simulink model "ENV"  (R2024b)
settings: Solver=FixedStepDiscrete  StartTime=0.0  StopTime=1  FixedStep=0.001  RelTol=1e-3  EnableMultiTasking=on
PreLoadFcn:
  | load('CAN_MESSAGE_bus.mat');
libraries: stm32blockslib x62, canmsglib x28, simulink x6, stm32f4xxblockslib x3
(part 1 of 5)
settings Model: DataDictionary=Master_Dictionary.sldd  EnableAccessToBaseWorkspace=off  STM32="{\"DigitalPortRead\":{\"ID\":\"ENV:1737\"},\"SPIControllerTransfer\":[{\"ID\":\"ENV:2145\"},{\"ID\":\"ENV:2146\"},{\"ID\":\"ENV:2312\"},{\"ID\":\"ENV:2313\"},{\"ID\":\"ENV:2314\"},{\"ID\":\"ENV:1806\"},{\"ID\":\"ENV:1805\"},{\"ID\":\"ENV:2392\"},{\"ID\":\"ENV:2393\"},{\"ID\":\"ENV:2419\"},{\"ID\":\"ENV:2421\"},{\"ID\":\"ENV:2432\"},{\"ID\":\"ENV:2439\"},{\"ID\":\"ENV:2451\"},{\"ID\":\"ENV:2458\"},{\"ID\":\"ENV:1834\"},{\"ID\":\"ENV:1835\"},{\"ID\":\"ENV:1851\"},{\"ID\":\"ENV:1852\"},{\"ID\":\"ENV:1875\"},{\"ID\":\"ENV:1876\"},{\"ID\":\"ENV:1893\"},{\"ID\":\"ENV:1894\"},{\"ID\":\"ENV:1915\"},{\"ID\":\"ENV:1916\"},{\"ID\":\"ENV:1940\"},{\"ID\":\"ENV:1941\"},{\"ID\":\"ENV:1960\"},{\"ID\":\"ENV:1961\"},{\"ID\":\"ENV:1982\"},{\"ID\":\"ENV:1983\"},{\"ID\":\"ENV:2003\"},{\"ID\":\"ENV:2004\"},{\"ID\":\"ENV:2024\"},{\"ID\":\"ENV:2025\"},{\"ID\":\"ENV:2071\"},{\"ID\":\"ENV:2072\"},{\"ID\":\"ENV:2091\"},{\"ID\":\"ENV:2092\"},{\"ID\":\"ENV:2117\"},{\"ID\":\"ENV:2118\"},{\"ID\":\"ENV:2169\"},{\"ID\":\"ENV:2170\"},{\"ID\":\"ENV:2191\"},{\"ID\":\"ENV:2192\"},{\"ID\":\"ENV:2213\"},{\"ID\":\"ENV:2214\"},{\"ID\":\"ENV:2234\"},{\"ID\":\"ENV:2235\"},{\"ID\":\"ENV:2254\"},{\"ID\":\"ENV:2255\"},{\"ID\":\"ENV:2522\"},{\"ID\":\"ENV:2521\"},{\"ID\":\"ENV:2520\"},{\"ID\":\"ENV:2519\"},{\"ID\":\"ENV:2518\"},{\"ID\":\"ENV:2517\"},{\"ID\":\"ENV:2516\"},{\"ID\":\"ENV:2515\"},{\"ID\":\"ENV:2549\"},{\"ID\":\"ENV:2550\"},{\"ID\":\"ENV:2555\"}],\"DigitalPortWrite\":[{\"ID\":\"ENV:2350\"},{\"ID\":\"ENV:2481\"}]}"  Creator=oxbro  LastModifiedBy=oxbro
settings SolverCC: AlgebraicLoopSolver=TrustRegion
settings DataIOCC: ReturnWorkspaceOutputs=off
settings OptimizationCC: DefaultParameterBehavior=Inlined  EnhancedBackFolding=on  PassReuseOutputArgsAs=Individual arguments  ZeroExternalMemoryAtStartup=off  ZeroInternalMemoryAtStartup=off  MaxStackSize=512  OptimizeBlockOrder=speed  DifferentSizesBufferReuse=on  OptimizationCustomize=off  EfficientTunableParamExpr=on
settings DebuggingCC: ParameterTunabilityLossMsg=error  UnconnectedInputMsg=warning  UnconnectedOutputMsg=warning  UnconnectedLineMsg=warning  ArithmeticOperatorsInVariantConditions=warning
settings HardwareCC: ProdBitPerPointer=32  ProdBitPerSizeT=32  ProdBitPerPtrDiffT=32  ProdLargestAtomicInteger=Long  ProdLargestAtomicFloat=Double  ProdWordSize=32  ProdLongLongMode=on  ProdHWDeviceType=ARM Compatible->ARM Cortex-M
settings ModelReferenceCC: EnableRefExpFcnMdlSchedulingChecks=on
settings SFSimCC: MATLABDynamicMemAlloc=off  CustomCodeUndefinedFunction=UseInterfaceOnly
settings RTWCC: Description=Embedded Coder  SystemTargetFile=ert.tlc  HardwareBoard=STM32H7xx Based (Single-core)  TemplateMakefile=ert_default_tmf  CustomHeaderCode="#include \"stm32h7xx_ll_tim.h\""  CustomInitializer=LL_TIM_EnableCounter(TIM2);  Toolchain=GNU Tools for ARM Embedded Processors  GPUComputeCapability=3.5
settings CodeAppCC: ForceParamTrailComments=on  IgnoreCustomStorageClasses=off  OperatorAnnotations=on  SimulinkDataObjDesc=on  SFDataObjDesc=on  InsertBlockDesc=on
settings ERTTargetCC: TargetLangStandard=C99 (ISO)  CodeReplacementLibrary=ARM Cortex-M  ExtModeTransport=3  ExtModeStaticAlloc=on  ExtModeStaticAllocSize=2048  ExtModeMexFile=ext_xcp  ExtModeIntrfLevel=Level2 - Open

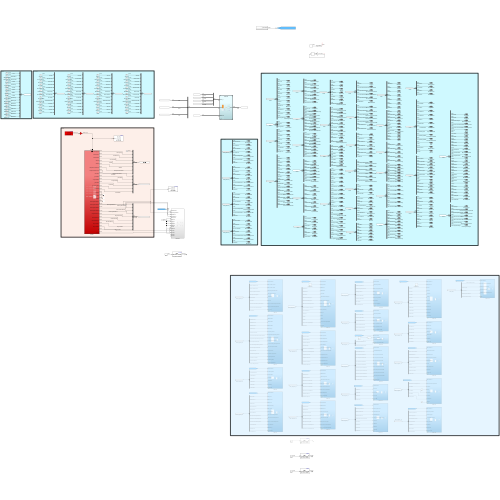
[thumbnail: Simulink's stored preview of the top-level diagram]
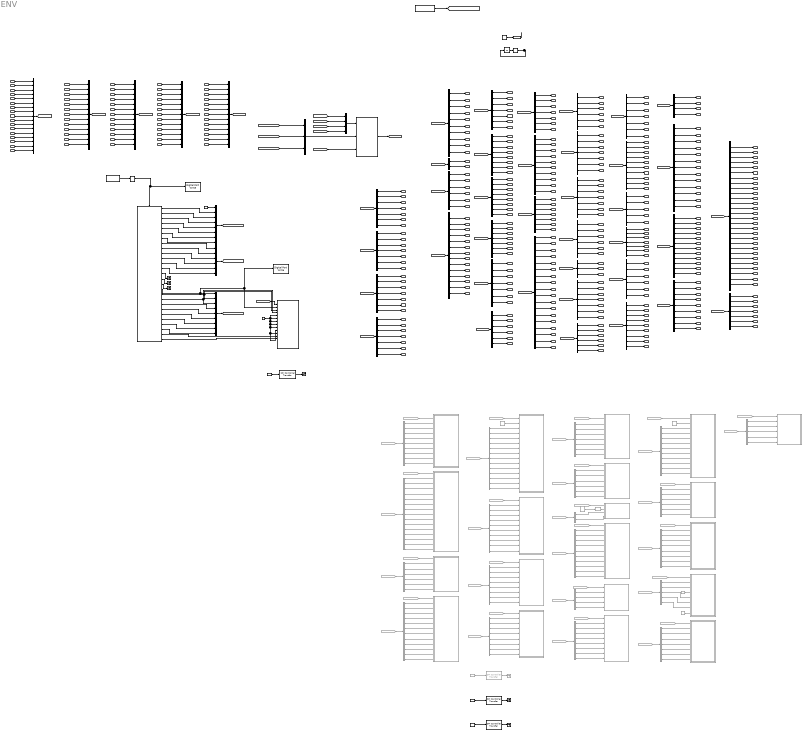
== system ENV ==
  note: CAN3
  note: CAN 1&2
  note: CAN4
  note: CAN1&2
  note: CAN3
  note: CAN3
  nMotorRL : Inport
  BInvDCOnRLIn : Inport  Port=2
  BInvErrorRL : Inport  Port=3
  BInvOnRLIn : Inport  Port=4
  BInvQuitDcOnRL : Inport  Port=5
  BQuitInvOnRL : Inport  Port=6
  BInvSysReadyRL : Inport  Port=7
  BInvWarnRL : Inport  Port=8
  MMotorMeasuredRL : Inport  Port=9
  NInvDTCRL : Inport  Port=10
  TMotorRL : Inport  Port=11
  VDCInvRL : Inport  Port=12
  TInvRL : Inport  Port=13
  nMotorRR : Inport  Port=14
  BInvDCOnRRIn : Inport  Port=15
  BInvErrorRR : Inport  Port=16
  BInvOnRRIn : Inport  Port=17
  BInvQuitDcOnRR : Inport  Port=18
  BQuitInvOnRR : Inport  Port=19
  BInvSysReadyRR : Inport  Port=20
  BInvWarnRR : Inport  Port=21
  MMotorMeasuredRR : Inport  Port=22
  NInvDTCRR : Inport  Port=23
  TMotorRR : Inport  Port=24
  VDCInvRR : Inport  Port=25
  TInvRR : Inport  Port=26
  nMotorFL : Inport  Port=27
  BInvDCOnFLIn : Inport  Port=28
  BInvErrorFL : Inport  Port=29
  BInvOnFLIn : Inport  Port=30
  BInvQuitDcOnFL : Inport  Port=31
  BQuitInvOnFL : Inport  Port=32
  BInvSysReadyFL : Inport  Port=33
  BInvWarnFL : Inport  Port=34
  MMotorMeasuredFL : Inport  Port=35
  NInvDTCFL : Inport  Port=36
  TMotorFL : Inport  Port=37
  VDCInvFL : Inport  Port=38
  TInvFL : Inport  Port=39
  nMotorFR : Inport  Port=40
  BInvDCOnFRIn : Inport  Port=41
  BInvErrorFR : Inport  Port=42
  BInvOnFRIn : Inport  Port=43
  BInvQuitDcOnFR : Inport  Port=44
  BQuitInvOnFR : Inport  Port=45
  BInvSysReadyFR : Inport  Port=46
  BInvWarnFR : Inport  Port=47
  MMotorMeasuredFR : Inport  Port=48
  NInvDTCFR : Inport  Port=49
  TMotorFR : Inport  Port=50
  VDCInvFR : Inport  Port=51
  TInvFR : Inport  Port=52
  IIVTS : Inport  Port=53
  IBMSHallEffect : Inport  Port=54
  VDCAccumulator : Inport  Port=55
  TCellMin : Inport  Port=56
  VCellAverage : Inport  Port=57
  VCellMax : Inport  Port=58
  TCellMax : Inport  Port=59
  IBMSDCL : Inport  Port=60
  VCellMin : Inport  Port=61
  RCellAverage : Inport  Port=62
  BBalancingOn : Inport  Port=63
  BBMSP0A0C : Inport  Port=64  OutDataTypeStr=boolean
  BBMSP0A0E : Inport  Port=65
  BBMSP0A10 : Inport  Port=66
  BBMSP0A80 : Inport  Port=67
  BBMSP0AC0 : Inport  Port=68
  BBMSP0AFA : Inport  Port=69
  Bus Creator : BusCreator  Inputs=3  OutDataTypeStr=Bus: CAN3Bus
  Bus Creator14 : BusCreator  Inputs=13  OutDataTypeStr=Bus: InverterFL
  Bus Creator15 : BusCreator  Inputs=13  OutDataTypeStr=Bus: InverterFR
  Bus Creator17 : BusCreator  Inputs=13  OutDataTypeStr=Bus: InverterRL
  Bus Creator18 : BusCreator  Inputs=17  OutDataTypeStr=Bus: BMS
  Bus Creator19 : BusCreator  Inputs=13  OutDataTypeStr=Bus: InverterRR
  Bus Creator2 : BusCreator  Inputs=8  OutDataTypeStr=Bus: DDU7
  Bus Creator3 : BusCreator  Inputs=6  OutDataTypeStr=Bus: IMU
      settings: InheritFromInputs=off
  Bus Creator4 : BusCreator  Inputs=9  OutDataTypeStr=Bus: STW
  Bus Selector : BusSelector  OutputSignals=TorqueControl.MFLFinal,TorqueControl.MFRFinal,TorqueControl.MRLFinal,TorqueControl.MRRFinal,BMSSignals.IIVTS,Systems.PActual,Systems.BBrakeError,Systems.BThrottleError,Systems.BOverpower,Limitations.BDischargeAllowed
  Bus Selector1 : BusSelector  OutputSignals=Systems.vChassis,Systems.PEnergyMeter
  Bus Selector10 : BusSelector  OutputSignals=TorqueControl.MTotalRequested,TorqueControl.rSlipRatioOptimal,TorqueControl.aCamberFL,TorqueControl.aCamberFR,TorqueControl.aCamberRL,TorqueControl.aCamberRR,TorqueControl.FTotalLateralLoadTransfer
  Bus Selector11 : BusSelector  OutputSignals=Systems.BTVOnEM,Systems.BTVOnOW,Systems.BDrivetrainCoolingOn,Systems.BDrivetrainCoolingOnEM,Systems.BDrivetrainCoolingOnOW,Systems.BTCOn,Systems.BTCOnEM,Systems.BTCOnOW,Systems.BEMSOn,Systems.BEMSOnEM,Systems.BEMSOnOW,Systems.BSpinningModeOn,Systems.BSpinningModeOnEM,Systems.BSpinningModeOnOW,Systems.rSOE,BMSSignals.BBalancingOn,BMSSignals.BBMSP0A0C,BMSSignals.BBMSP0A0E,BMSSignals.BBMSP0A10,BMSSignals.BBMSP0A80,BMSSignals.BBMSP0AC0,BMSSignals.BBMSP0AFA,TorqueControl.NLap,Systems.NEventMode,Systems.rTorqueSplit,Systems.NThrottleMap,Systems.NThrottleMapEM,Systems.NThrottleMapOW
  Bus Selector12 : BusSelector  OutputSignals=Systems.aSteeringAngle,Limitations.PLowCellVoltageDischargeDerate,Limitations.PHighCellVoltageRegenDerate,TorqueControl.MDriverDischargeRequested,TorqueControl.MDriverRegenRequested,TorqueControl.PPCIntegralTermDischarge,TorqueControl.PPCIntegralTermRegen
  Bus Selector13 : BusSelector  OutputSignals=Stateflow.NInvState,Systems.BInverterErrorRear,Systems.BInverterErrorFront,Systems.BErrorReset,InverterSignals.InverterRLSignals.TInvRL,InverterSignals.InverterFRSignals.TMotorFR,BMSSignals.VDCAccumulator,TorqueControl.EBudget,TorqueControl.BTVOK,TorqueControl.sSector
  Bus Selector14 : BusSelector  OutputSignals=Systems.sChassis,Limitations.PInvTemperatureDerate,Limitations.PInvTemperatureDerateFR,Limitations.PInvTemperatureDerateFL,Limitations.PInvTemperatureDerateRR,BMSSignals.IBMSHallEffect
  Bus Selector15 : BusSelector  OutputSignals=TorqueControl.NABSMultiplierRR,TorqueControl.MTractionControlRRTotal,TorqueControl.MTotalFinal,TorqueControl.rSlipRatioFLActual,TorqueControl.rSlipRatioFRActual,TorqueControl.rSlipRatioRLActual,TorqueControl.FTyreVerticalFR
  Bus Selector16 : BusSelector  Commented=on  OutputSignals=SystemsBus.BEncoderErrorFront,SystemsBus.BEncoderErrorRear,SystemsBus.BSpinningModelActivated,TorqueControlBus.BTorqueVectoringOK,TorqueControlBus.MTotalFinal,SystemsBus.PActual,TorqueControlBus.PPowerControllerProportionalTerm,TorqueControlBus.PPowerControllerIntegralTerm,SystemsBus.vChassis
  Bus Selector17 : BusSelector  Commented=on  OutputSignals=BMSSignalsBus.BBMSP0A80,BMSSignalsBus.BBMSP0AC0,BMSSignalsBus.BBMSP0AFA,SystemsBus.PDischarge,LimitationsBus.rDischargeDerate,LimitationsBus.rHighCellTemperatureDischargeDerate,LimitationsBus.rHighCellTemperatureRegenDerate,LimitationsBus.rInvTemperatureDerate,LimitationsBus.rLowCellVoltageDischargeDerate,LimitationsBus.rMotorTemperatureDerate,LimitationsBus.rRegenDerate,LimitationsBus.rSOCDischargeDerate,LimitationsBus.rSOCRegenDerate,TorqueControlBus.rSOCTargetError,LimitationsBus.rSpeedRegenDerate
  Bus Selector18 : BusSelector  OutputSignals=Systems.PDischargeMax,Systems.PDischargeMaxEM,Systems.PDischargeMaxOW,Systems.PEngineBraking,Systems.PEngineBrakingEM,Systems.PEngineBrakingOW,Systems.rGrip,Systems.EOffset,Systems.NTCKdSelector,Systems.NPCKpSelector,Systems.MRegenMax,Systems.rTorqueSplitEM
  Bus Selector19 : BusSelector  OutputSignals=Systems.tThrottleError,TorqueControl.MTorqueDistributionRR,TorqueControl.NTractionControlMultiplierRL,TorqueControl.NTractionControlMultiplierRR,TorqueControl.NABSMultiplierFL,TorqueControl.NABSMultiplierFR,TorqueControl.NABSMultiplierRL,TorqueControl.FTyreVerticalFL
  Bus Selector2 : BusSelector  OutputSignals=WheelSpeeds.vWheelFL,WheelSpeeds.vWheelFR,InverterSignals.InverterFLSignals.nMotorFL,InverterSignals.InverterFRSignals.nMotorFR,Systems.rThrottlePedal1,Systems.BPageUp,InverterSignals.InverterRLSignals.BQuitInvOnRL,InverterSignals.InverterFLSignals.BQuitInvOnFL,InverterSignals.InverterRRSignals.BQuitInvOnRR,InverterSignals.InverterFRSignals.BQuitInvOnFR,Stateflow.BInvErrorResetRL,Stateflow.BInvErrorResetRR,Stateflow.BInvErrorResetFL,Stateflow.BInvErrorResetFR
  Bus Selector20 : BusSelector  OutputSignals=Stateflow.BInvDCOnRLOut,Stateflow.BInvEnableRL,Stateflow.BInvErrorResetRL,Stateflow.BInvOnRLOut,Stateflow.MTorqueLimitNegativeRL,Stateflow.MTorqueLimitPositiveRL,TorqueControl.MRLFinal
  Bus Selector21 : BusSelector  OutputSignals=Stateflow.BInvDCOnFLOut,Stateflow.BInvEnableFL,Stateflow.BInvErrorResetFL,Stateflow.BInvOnFLOut,Stateflow.MTorqueLimitNegativeFL,Stateflow.MTorqueLimitPositiveFL,TorqueControl.MFLFinal
  Bus Selector22 : BusSelector  OutputSignals=Stateflow.BInvDCOnRROut,Stateflow.BInvEnableRR,Stateflow.BInvErrorResetRR,Stateflow.BInvOnRROut,Stateflow.MTorqueLimitNegativeRR,Stateflow.MTorqueLimitPositiveRR,TorqueControl.MRRFinal
  Bus Selector23 : BusSelector  OutputSignals=Stateflow.BInvDCOnFROut,Stateflow.BInvEnableFR,Stateflow.BInvErrorResetFR,Stateflow.BInvOnFROut,Stateflow.MTorqueLimitNegativeFR,Stateflow.MTorqueLimitPositiveFR,TorqueControl.MFRFinal
  Bus Selector24 : BusSelector  OutputSignals=Systems.tBrakeError,TorqueControl.nYawRateErrorActual,TorqueControl.MTorqueDistributionRL,TorqueControl.MTractionControlRLTotal,TorqueControl.MTractionControlFRTotal,TorqueControl.MTractionControlFLTotal,TorqueControl.rSlipRatioRRActual
  Bus Selector25 : BusSelector  Commented=on  OutputSignals=SensorSignalsBus.VDamperPotentiometerFL,SensorSignalsBus.VDamperPotentiometerFR
  Bus Selector26 : BusSelector  Commented=on  OutputSignals=TorqueControlBus.MTotalEMSRequested,LimitationsBus.rInvTemperatureDerateFL,LimitationsBus.rInvTemperatureDerateFR,LimitationsBus.rInvTemperatureDerateRL,LimitationsBus.rInvTemperatureDerateRR,LimitationsBus.rMotorTemperatureDerateFL,LimitationsBus.rMotorTemperatureDerateFR,LimitationsBus.rMotorTemperatureDerateRL,LimitationsBus.rMotorTemperatureDerateRR,SystemsBus.rThrottlePedal
  Bus Selector27 : BusSelector  Commented=on  OutputSignals=InverterSignalsBus.InverterFLSignalsBus.nMotorFL,InverterSignalsBus.InverterFRSignalsBus.nMotorFR,InverterSignalsBus.InverterRLSignalsBus.nMotorRL,InverterSignalsBus.InverterRRSignalsBus.nMotorRR
  Bus Selector28 : BusSelector  Commented=on  OutputSignals=LimitationsBus.BDischargeAllowed,SystemsBus.BEMS1000mPoint,SystemsBus.BEMS995mPoint,TorqueControlBus.MDriverDischargeRequested,TorqueControlBus.MFLFinal,TorqueControlBus.MFRFinal,TorqueControlBus.MRLFinal,TorqueControlBus.MRRFinal
  Bus Selector29 : BusSelector  OutputSignals=Stateflow.NCarState,Systems.pBrakeF,Systems.pBrakeR,Systems.tAppsTimer,BMSSignals.VCellMax,BMSSignals.VCellMin,Limitations.PSOCDischargeDerate
  Bus Selector3 : BusSelector  OutputSignals=WheelSpeeds.vWheelRL,WheelSpeeds.vWheelRR,InverterSignals.InverterRLSignals.nMotorRL,InverterSignals.InverterRRSignals.nMotorRR,Systems.rThrottlePedal,Systems.BPageDown
  Bus Selector30 : BusSelector  OutputSignals=Limitations.rSpeedRegenDerateRL,Limitations.rSpeedRegenDerateFR,Limitations.rSpeedRegenDerateFL,Limitations.BSpeedDerateOn,Limitations.PDischargeDerate,Limitations.PRegenDerate,TorqueControl.PRegenRequested,TorqueControl.PDischargeLimit,TorqueControl.PRegenLimit,TorqueControl.PPCDischargeRequested
  Bus Selector31 : BusSelector  OutputSignals=Systems.BPCComplete,Systems.BBrakeLight,Stateflow.BReadyToDriveBuzzer,Systems.BAccuFanOn,Systems.BMotorRBHFanOn,Systems.BInverterFanOn,Systems.BInvLVOn
  Bus Selector32 : BusSelector  Commented=on  OutputSignals=InverterSignalsBus.InverterFLSignalsBus.TInvFL,InverterSignalsBus.InverterFRSignalsBus.TInvFR,SystemsBus.TInvMax,InverterSignalsBus.InverterRLSignalsBus.TInvRL,InverterSignalsBus.InverterRRSignalsBus.TInvRR,InverterSignalsBus.InverterFLSignalsBus.TMotorFL,InverterSignalsBus.InverterFRSignalsBus.TMotorFR,SystemsBus.TMotorMax,InverterSignalsBus.InverterRLSignalsBus.TMotorRL,InverterSignalsBus.InverterRRSignalsBus.TMotorRR
  Bus Selector33 : BusSelector  OutputSignals=Systems.TMotorMax,Systems.TInvMax,InverterSignals.InverterRLSignals.TMotorRL,InverterSignals.InverterRLSignals.VDCInvRL,InverterSignals.InverterRRSignals.TMotorRR,InverterSignals.InverterFLSignals.TMotorFL
  Bus Selector34 : BusSelector  OutputSignals=TorqueControl.ETotalRequested,TorqueControl.ESector1Remaining,TorqueControl.ESector2Remaining,TorqueControl.ESector3Remaining,TorqueControl.ESector4Remaining
  Bus Selector35 : BusSelector  OutputSignals=TorqueControl.ERemaining,TorqueControl.FTotalDownforce,TorqueControl.aCamberGainRollF,TorqueControl.aCamberGainRollR,TorqueControl.aCamberGainHeaveF,TorqueControl.aCamberGainHeaveR,TorqueControl.aRollAngle
  Bus Selector36 : BusSelector  Commented=on  OutputSignals=InverterSignalsBus.InverterFLSignalsBus.NInvDTCFL,InverterSignalsBus.InverterFRSignalsBus.NInvDTCFR,InverterSignalsBus.InverterRLSignalsBus.NInvDTCRL,InverterSignalsBus.InverterRRSignalsBus.NInvDTCRR,BMSSignalsBus.TCellMax,BMSSignalsBus.VCellDelta
  Bus Selector37 : BusSelector  Commented=on  OutputSignals=SystemsBus.BAccumulatorFanOn,SystemsBus.BEMSActivated,SystemsBus.BTractionControlActivated,BMSSignalsBus.IBMSHallEffect,BMSSignalsBus.IIVTS,TorqueControlBus.MTotalRequested,BMSSignalsBus.VDCAccumulator,InverterSignalsBus.InverterRLSignalsBus.VDCInvRL
  Bus Selector38 : BusSelector  OutputSignals=TorqueControl.NSectorGlobal,TorqueControl.NSectorLap,TorqueControl.NSector3Remaining,TorqueControl.NSector4Remaining,TorqueControl.NSector5Remaining,TorqueControl.NSector6Remaining,TorqueControl.NSector7Remaining,TorqueControl.NSector8Remaining,TorqueControl.ESector8Remaining
  Bus Selector39 : BusSelector  Commented=on  OutputSignals=SystemsBus.NTractionControlKpSelector,BMSSignalsBus.TCellMin,BMSSignalsBus.VCellMax,BMSSignalsBus.VCellMin,SensorSignalsBus.VLVSystem
  Bus Selector4 : BusSelector  OutputSignals=Systems.tPedalOverlap,TorqueControl.PPCProportionalTermDischarge,TorqueControl.MPCDischargeRequested,TorqueControl.PPCProportionalTermRegen,TorqueControl.MPCRegenRequested,TorqueControl.MDischargeLimited,TorqueControl.NTractionControlMultiplierFL,TorqueControl.NTractionControlMultiplierFR
  Bus Selector40 : BusSelector  Commented=on  OutputSignals=TorqueControlBus.PDischargeLimited,SystemsBus.aSteeringAngle,TorqueControlBus.nYawRateErrorActual,SystemsBus.rRegenPaddle,TorqueControlBus.rSplitRear,SystemsBus.tAppsTimer,SystemsBus.tPedalOverlap
  Bus Selector41 : BusSelector  Commented=on  OutputSignals=TorqueControlBus.rSOETargetError,SystemsBus.sEMS1000m,WheelSpeedsBus.vWheelFL,WheelSpeedsBus.vWheelFR,WheelSpeedsBus.vWheelRL,WheelSpeedsBus.vWheelRR
  Bus Selector42 : BusSelector  OutputSignals=Limitations.PInvTemperatureDerateRL,Limitations.PMotorTemperatureDerate,Limitations.PMotorTemperatureDerateFR,Limitations.PMotorTemperatureDerateFL,Limitations.PMotorTemperatureDerateRR,TorqueControl.aCamberGainSteerFL,TorqueControl.aCamberGainSteerFR
  Bus Selector43 : BusSelector  Commented=on  OutputSignals=SystemsBus.BAccumulatorFanOn,SystemsBus.BBrakeLight,SystemsBus.BInvLVOn,StateflowBus.BReadyToDriveBuzzer,SystemsBus.BAccumulatorFanDuty
  Bus Selector44 : BusSelector  Commented=on  OutputSignals=SystemsBus.BAppsOK,SystemsBus.BBrakeError,SystemsBus.BBrakeOn,SystemsBus.BPedalOverlap,SystemsBus.BRegenOn,SystemsBus.BThrottleError,SystemsBus.BTorqueVectoringActivated,TorqueControlBus.MPowerControllerRequested,TorqueControlBus.PPowerControllerRequested,SystemsBus.rThrottlePedal,SystemsBus.tBrakeError,SystemsBus.tThrottleError
  Bus Selector45 : BusSelector  Commented=on  OutputSignals=StateflowBus.BReadyToDrive,TorqueControlBus.NABSMultiplierRL,TorqueControlBus.NABSMultiplierRR,SystemsBus.NThrottleMap,TorqueControlBus.NTractionControlMultiplierRL,TorqueControlBus.NTractionControlMultiplierRR,TorqueControlBus.rSlipRatioFLActual,TorqueControlBus.rSlipRatioFRActual,TorqueControlBus.rSlipRatioRLActual,TorqueControlBus.rSlipRatioRRActual
  Bus Selector46 : BusSelector  Commented=on  OutputSignals=BMSSignalsBus.NBMSDLC,StateflowBus.NBMSState,StateflowBus.NInvState,SystemsBus.NModeNumberDisplay5,SystemsBus.NModeNumberDisplay6,SystemsBus.NPowerControllerKpSelector,SystemsBus.NTorqueSplitSpeedSelector,SystemsBus.PEngineBraking,SystemsBus.PRegen,SystemsBus.rSOC,SystemsBus.rSOE,SystemsBus.rTorqueVectoringMultiplier,SystemsBus.sChassis
  Bus Selector47 : BusSelector  OutputSignals=Limitations.PMotorTemperatureDerateRL,Limitations.PTSTemperatureDerateFR,Limitations.PTSTemperatureDerateFL,Limitations.PTSTemperatureDerateRR,Limitations.PTSTemperatureDerateRL,Limitations.PHighCellTemperatureDerate
  Bus Selector48 : BusSelector  OutputSignals=TorqueControl.ESector,TorqueControl.xHeaveTravelF,TorqueControl.xHeaveTravelR
  Bus Selector49 : BusSelector  OutputSignals=Stateflow.NBMSState,InverterSignals.InverterRRSignals.TInvRR,InverterSignals.InverterFLSignals.TInvFL,InverterSignals.InverterFRSignals.TInvFR,BMSSignals.TCellMax,BMSSignals.TCellMin,TorqueControl.rSplitRear
  Bus Selector5 : BusSelector  OutputSignals=Systems.pBrakeMax,Systems.rRegenPaddle,Systems.xDamperFL,Systems.xDamperFR,Systems.xDamperRL,Systems.xDamperRR,Systems.BIMUOK,Systems.tIMUError,Systems.BDataMark
  Bus Selector50 : BusSelector  Commented=on  OutputSignals=BMSSignalsBus.BBMSP0A0C,BMSSignalsBus.BBalancingActive,TorqueControlBus.MTractionControlFLTotal,TorqueControlBus.MTractionControlFRTotal,TorqueControlBus.MTractionControlRLTotal,TorqueControlBus.MTractionControlRRTotal,TorqueControlBus.NABSMultiplierFL,TorqueControlBus.NABSMultiplierFR
  Bus Selector51 : BusSelector  Commented=on  OutputSignals=BMSSignalsBus.BBMSP0A0E,BMSSignalsBus.BBMSP0A10,TorqueControlBus.MTorqueVectoringFL,TorqueControlBus.MTorqueVectoringFR,TorqueControlBus.MTorqueVectoringRL,TorqueControlBus.MTorqueVectoringRR,TorqueControlBus.NTractionControlMultiplierFL,TorqueControlBus.NTractionControlMultiplierFR
  Bus Selector52 : BusSelector  Commented=on  OutputSignals=TorqueControlBus.MDischargeLimited,TorqueControlBus.MDriverRegenRequested,TorqueControlBus.MRegenLimited,TorqueControlBus.MSpinningModelFL,TorqueControlBus.MSpinningModelFR,StateflowBus.NCarState,TorqueControlBus.rSlipRatioOptimal
  Bus Selector53 : BusSelector  OutputSignals=TorqueControl.ESector9Remaining,TorqueControl.ESector10Remaining,TorqueControl.ESector11Remaining,TorqueControl.ESector12Remaining,TorqueControl.NSector1Remaining,TorqueControl.NSector2Remaining
  Bus Selector54 : BusSelector  OutputSignals=TorqueControl.NSector9Remaining,TorqueControl.NSector10Remaining,TorqueControl.NSector11Remaining,TorqueControl.NSector12Remaining,TorqueControl.ESector5Remaining,TorqueControl.ESector6Remaining,TorqueControl.ESector7Remaining
  Bus Selector55 : BusSelector  OutputSignals=Systems.rTorqueSplitOW,Systems.PRegenMax,Systems.PRegenMaxEM,Systems.PRegenMaxOW,Systems.rTVMultiplier,Systems.rTVMultiplierEM,Systems.rTVMultiplierOW,Systems.rEngineBrakingSplit,Systems.rEngineBrakingSplitEM,Systems.rEngineBrakingSplitOW,Systems.rSOC,Stateflow.BReadyToDrive,Systems.BTVOn
  Bus Selector56 : BusSelector  Commented=on  OutputSignals=TorqueControlBus.MSpinningModelRL,TorqueControlBus.MSpinningModelRR,TorqueControlBus.MTorqueDistributionFL,TorqueControlBus.MTorqueDistributionFR,TorqueControlBus.MTorqueDistributionRL,TorqueControlBus.MTorqueDistributionRR
  Bus Selector6 : BusSelector  OutputSignals=TorqueControl.FTyreVerticalRL,TorqueControl.FTyreVerticalRR,TorqueControl.aSlipAngleFL,TorqueControl.aSlipAngleFR,TorqueControl.aSlipAngleRL,TorqueControl.aSlipAngleRR
  Bus Selector7 : BusSelector  OutputSignals=InverterSignals.InverterRLSignals.NInvDTCRL,InverterSignals.InverterRRSignals.NInvDTCRR,InverterSignals.InverterFLSignals.NInvDTCFL,InverterSignals.InverterFRSignals.NInvDTCFR
  Bus Selector8 : BusSelector  OutputSignals=Systems.BBrakeOn,Systems.BPedalOverlap,Systems.BAppsOK,Systems.BRegenOn,Systems.BxDamperFLOk,Systems.BxDamperFROk,Systems.BxDamperRLOk,Systems.BxDamperRROk,Systems.BIMUError,Systems.BCalibrationOn,Limitations.PSOCRegenDerate,Limitations.rSpeedRegenDerateRR,TorqueControl.PPCRegenRequested,TorqueControl.PDischargeLimited,TorqueControl.BEMSDriverSignal1,TorqueControl.BEMSDriverSignal2,TorqueControl.BEMSDriverSignal3,TorqueControl.FLongitudinalLoadTransfer
  Bus Selector9 : BusSelector  OutputSignals=TorqueControl.MTorqueVectoringFL,TorqueControl.MTorqueVectoringFR,TorqueControl.MTorqueVectoringRL,TorqueControl.MTorqueVectoringRR,TorqueControl.MTorqueDistributionFL,TorqueControl.MTorqueDistributionFR,TorqueControl.MRegenLimited
  CAN Rx : Subsystem  TreatAsAtomicUnit=on
  CAN Tx : Subsystem  Commented=on
  CAN Tx1 : Subsystem  Commented=on
  CAN Tx10 : Subsystem  Commented=on
  CAN Tx11 : Subsystem  Commented=on
  CAN Tx12 : Subsystem  Commented=on
  CAN Tx13 : Subsystem  Commented=on
  CAN Tx14 : Subsystem  Commented=on
  CAN Tx15 : Subsystem  Commented=on
  CAN Tx16 : Subsystem  Commented=on
  CAN Tx17 : Subsystem  Commented=on
  CAN Tx18 : Subsystem  Commented=on
  CAN Tx19 : Subsystem  Commented=on
  CAN Tx2 : Subsystem  Commented=on
  CAN Tx20 : Subsystem
  CAN Tx3 : Subsystem  Commented=on
  CAN Tx4 : Subsystem  Commented=on
  CAN Tx5 : Subsystem  Commented=on
  CAN Tx6 : Subsystem  Commented=on
  CAN Tx7 : Subsystem  Commented=on
  CAN Tx8 : Subsystem  Commented=on
  CAN Tx9 : Subsystem  Commented=on
  CAN1_2Bus : BusCreator  Inputs=4  OutDataTypeStr=Bus: CAN1_2Bus
  Compare To Constant : simulink/Logic and Bit Operations/Compare To Constant  relop=>=  const=125  OutDataTypeStr=boolean
  Constant : Constant  Commented=on  Value=92
  Constant1 : Constant  Commented=on  Value=92
  Constant2 : Constant  Value=69
  Constant3 : Constant
  Counter Free-Running : simulink/Sources/Counter Free-Running  Commented=on  NumBits=16  tsamp=-1
  Counter Limited : simulink/Sources/Counter Limited  uplimit=250  tsamp=-1
  Data Type Conversion : DataTypeConversion  Commented=on  OutDataTypeStr=uint16  SaturateOnIntegerOverflow=off  RndMeth=Floor
  Digital Port Read1 : stm32f4xxblockslib/Digital Port Read  PortName=GPIOA  PinNumber=2  ReadOperation=on  IOAsArray=off  SampleTime=-1  EnableSimPort=off  hoistedMaskSrc=ECSoC/ECSimCodegen/Digital Port Read
      settings: LibrarySourceBlock=stm32f2xxblockslib/Digital Port Read
  Digital Port Write : stm32f4xxblockslib/Digital Port Write  PortName=GPIOB  PinNumber=4  ReadOperation=off  IOAsArray=off  EnableSimPort=off  hoistedMaskSrc=ECSoC/ECSimCodegen/Digital Port Write
      settings: LibrarySourceBlock=stm32h7xxblockslib/Digital Port Write
  Digital Port Write1 : stm32f4xxblockslib/Digital Port Write  PortName=GPIOB  PinNumber=5  ReadOperation=off  IOAsArray=off  EnableSimPort=off  hoistedMaskSrc=ECSoC/ECSimCodegen/Digital Port Write
      settings: LibrarySourceBlock=stm32h7xxblockslib/Digital Port Write
  Etas_Signals_01 : From  Commented=on  GotoTag=Global
  Etas_Signals_02 : From  Commented=on  GotoTag=Global
  Etas_Signals_03 : From  Commented=on  GotoTag=Global
  Etas_Signals_04 : From  Commented=on  GotoTag=Global
  Etas_Signals_05 : From  Commented=on  GotoTag=Global
  Etas_Signals_06 : From  Commented=on  GotoTag=Global
  Etas_Signals_07 : From  Commented=on  GotoTag=Global
  Etas_Signals_08 : From  Commented=on  GotoTag=Global
  Etas_Signals_09 : From  Commented=on  GotoTag=Global
  Etas_Signals_{10..19} (10 alike) : From  Commented=on  GotoTag=Global
  From{51..70} (20 alike) : From  Commented=on  GotoTag=MCPInitialized
  Model : ModelReference  ModelNameDialog=MASTER.slx  SimulationMode=Normal  ModelReferenceVersion=13.6
  Multiplexer1? : simulink/Sources/Counter Limited  Commented=on  uplimit=1  tsamp=-1
  Multiplexer? : simulink/Sources/Counter Limited  Commented=on  uplimit=1  tsamp=-1
  NOT : Logic  Operator=NOT  IconShape=distinctive  AllPortsSameDT=off  OutDataTypeStr=boolean
  NOT4 : Logic  Operator=NOT  IconShape=distinctive  AllPortsSameDT=off  OutDataTypeStr=boolean
  PDM_Req : From  Commented=on  GotoTag=Global
  RTS1 : Constant  Value=0x84  OutDataTypeStr=uint8  SampleTime=-1
  RTS2 : Constant  Commented=on  Value=0x81  OutDataTypeStr=uint8  SampleTime=-1
  RTS3 : Constant  Value=0x81  OutDataTypeStr=uint8  SampleTime=-1
  RTS4 : Constant  Value=0x82  OutDataTypeStr=uint8  SampleTime=-1
  SPI Controller Transfer1 : stm32blockslib/SPI Controller Transfer  Priority=2  SPIModuleSelect=SPI1  ClockPolarity=Low  ClockPhase=1 Edge  SPIModule=uint32(0)  Mode=Master  BusSpeed=uint32(1000000)  FirstBitToTransfer=Most significant bit (MSB)  ClockMode=0  BlockFunction=Transfer  EnableRegisterAddress=off  RegisterAddress=0  OutputDataType=uint8  OutputDataLength=1  OutputStatus=off  BlockingMode=off  Timeout=0.01  DataBits=8  UseCustomSSPin=Explicit GPIO calls  ActiveLowSSPin=Active low  Port_Select=GPIOA  Pin=1
      settings: LibrarySourceBlock=stm32h7xxblockslib/SPI Controller Transfer
  SPI Controller Transfer2 : stm32blockslib/SPI Controller Transfer  Priority=2  SPIModuleSelect=SPI1  ClockPolarity=Low  ClockPhase=1 Edge  SPIModule=uint32(0)  Mode=Master  BusSpeed=uint32(1000000)  FirstBitToTransfer=Most significant bit (MSB)  ClockMode=0  BlockFunction=Transfer  EnableRegisterAddress=off  RegisterAddress=0  OutputDataType=uint8  OutputDataLength=1  OutputStatus=off  BlockingMode=off  Timeout=0.01  DataBits=8  UseCustomSSPin=Explicit GPIO calls  ActiveLowSSPin=Active low  Port_Select=GPIOA  Pin=4
      settings: LibrarySourceBlock=stm32h7xxblockslib/SPI Controller Transfer
  SPI Controller Transfer3 : stm32blockslib/SPI Controller Transfer  Priority=2  Commented=on  SPIModuleSelect=SPI1  ClockPolarity=Low  ClockPhase=1 Edge  SPIModule=uint32(0)  Mode=Master  BusSpeed=uint32(1000000)  FirstBitToTransfer=Most significant bit (MSB)  ClockMode=0  BlockFunction=Transfer  EnableRegisterAddress=off  RegisterAddress=0  OutputDataType=uint8  OutputDataLength=1  OutputStatus=off  BlockingMode=off  Timeout=0.01  DataBits=8  UseCustomSSPin=Explicit GPIO calls  ActiveLowSSPin=Active low  Port_Select=GPIOA  Pin=4
      settings: LibrarySourceBlock=stm32h7xxblockslib/SPI Controller Transfer
  SPI Controller Transfer5 : stm32blockslib/SPI Controller Transfer  Priority=2  SPIModuleSelect=SPI1  ClockPolarity=Low  ClockPhase=1 Edge  SPIModule=uint32(0)  Mode=Master  BusSpeed=uint32(1000000)  FirstBitToTransfer=Most significant bit (MSB)  ClockMode=0  BlockFunction=Transfer  EnableRegisterAddress=off  RegisterAddress=0  OutputDataType=uint8  OutputDataLength=1  OutputStatus=off  BlockingMode=off  Timeout=0.01  DataBits=8  UseCustomSSPin=Explicit GPIO calls  ActiveLowSSPin=Active low  Port_Select=GPIOA  Pin=4
      settings: LibrarySourceBlock=stm32h7xxblockslib/SPI Controller Transfer
  Subsystem : Subsystem
  Terminator{,1..3,5..6} (6 alike) : Terminator
  Terminator4 : Terminator  Commented=on
  Unit Delay : UnitDelay  SampleTime=-1  HasFrameUpgradeWarning=on
  BInvDCOnRLOut : Outport  VectorParamsAs1DForOutWhenUnconnected=off
  BInvEnableRL : Outport  Port=2  VectorParamsAs1DForOutWhenUnconnected=off
  BInvErrorResetRL : Outport  Port=3  VectorParamsAs1DForOutWhenUnconnected=off
  BInvOnRLOut : Outport  Port=4  VectorParamsAs1DForOutWhenUnconnected=off
  MTorqueLimitNegativeRL : Outport  Port=5  VectorParamsAs1DForOutWhenUnconnected=off
  MTorqueLimitPositiveRL : Outport  Port=6  VectorParamsAs1DForOutWhenUnconnected=off
  MInvRLFinal : Outport  Port=7  VectorParamsAs1DForOutWhenUnconnected=off
  BInvDCOnFLOut : Outport  Port=8  VectorParamsAs1DForOutWhenUnconnected=off
  BInvEnableFL : Outport  Port=9  VectorParamsAs1DForOutWhenUnconnected=off
  BInvErrorResetFL : Outport  Port=10  VectorParamsAs1DForOutWhenUnconnected=off
  BInvOnFLOut : Outport  Port=11  VectorParamsAs1DForOutWhenUnconnected=off
  MTorqueLimitNegativeFL : Outport  Port=12  VectorParamsAs1DForOutWhenUnconnected=off
  MTorqueLimitPositiveFL : Outport  Port=13  VectorParamsAs1DForOutWhenUnconnected=off
  MInvFLFinal : Outport  Port=14  VectorParamsAs1DForOutWhenUnconnected=off
  BInvDCOnRROut : Outport  Port=15  VectorParamsAs1DForOutWhenUnconnected=off
  BInvEnableRR : Outport  Port=16  VectorParamsAs1DForOutWhenUnconnected=off
  BInvErrorResetRR : Outport  Port=17  VectorParamsAs1DForOutWhenUnconnected=off
  BInvOnRROut : Outport  Port=18  VectorParamsAs1DForOutWhenUnconnected=off
  MTorqueLimitNegativeRR : Outport  Port=19  VectorParamsAs1DForOutWhenUnconnected=off
  MTorqueLimitPositiveRR : Outport  Port=20  VectorParamsAs1DForOutWhenUnconnected=off
  MInvRRFinal : Outport  Port=21  VectorParamsAs1DForOutWhenUnconnected=off
  BInvDCOnFROut : Outport  Port=22  VectorParamsAs1DForOutWhenUnconnected=off
  BInvEnableFR : Outport  Port=23  VectorParamsAs1DForOutWhenUnconnected=off
  BInvErrorResetFR : Outport  Port=24  VectorParamsAs1DForOutWhenUnconnected=off
  BInvOnFROut : Outport  Port=25  VectorParamsAs1DForOutWhenUnconnected=off
  MTorqueLimitNegativeFR : Outport  Port=26  VectorParamsAs1DForOutWhenUnconnected=off
  MTorqueLimitPositiveFR : Outport  Port=27  VectorParamsAs1DForOutWhenUnconnected=off
  MInvFRFinal : Outport  Port=28  VectorParamsAs1DForOutWhenUnconnected=off
  MTotalFinal : Outport  Port=29  VectorParamsAs1DForOutWhenUnconnected=off
  PActual : Outport  Port=30  VectorParamsAs1DForOutWhenUnconnected=off
  rSpeedRegenDerateRR : Outport  Port=31  VectorParamsAs1DForOutWhenUnconnected=off
  PDischargeMax : Outport  Port=32  VectorParamsAs1DForOutWhenUnconnected=off
  rThrottlePedal : Outport  Port=33  VectorParamsAs1DForOutWhenUnconnected=off
  rThrottlePedal1 : Outport  Port=34  VectorParamsAs1DForOutWhenUnconnected=off
  aSteeringAngle : Outport  Port=35  VectorParamsAs1DForOutWhenUnconnected=off
  pBrakeF : Outport  Port=36  VectorParamsAs1DForOutWhenUnconnected=off
  pBrakeR : Outport  Port=37  VectorParamsAs1DForOutWhenUnconnected=off
  BBMSP0A80Out : Outport  Port=38  VectorParamsAs1DForOutWhenUnconnected=off
  BBMSP0AC0Out : Outport  Port=39  VectorParamsAs1DForOutWhenUnconnected=off
  BBMSP0AFAOut : Outport  Port=40  VectorParamsAs1DForOutWhenUnconnected=off
  BBMSP0A0COut : Outport  Port=41  VectorParamsAs1DForOutWhenUnconnected=off
  BBMSP0A0EOut : Outport  Port=42  VectorParamsAs1DForOutWhenUnconnected=off
  BBMSP0A10Out : Outport  Port=43  VectorParamsAs1DForOutWhenUnconnected=off
  BTVOK : Outport  Port=44  VectorParamsAs1DForOutWhenUnconnected=off
  NInvDTCRROut : Outport  Port=45  VectorParamsAs1DForOutWhenUnconnected=off
  NInvDTCRLOut : Outport  Port=46  VectorParamsAs1DForOutWhenUnconnected=off
  NInvDTCFROut : Outport  Port=47  VectorParamsAs1DForOutWhenUnconnected=off
  NInvDTCFLOut : Outport  Port=48  VectorParamsAs1DForOutWhenUnconnected=off
  IIVTSOut : Outport  Port=49  VectorParamsAs1DForOutWhenUnconnected=off
  MFRFinal : Outport  Port=50  VectorParamsAs1DForOutWhenUnconnected=off
  MFLFinal : Outport  Port=51  VectorParamsAs1DForOutWhenUnconnected=off
  MRLFinal : Outport  Port=52  VectorParamsAs1DForOutWhenUnconnected=off
  MRRFinal : Outport  Port=53  VectorParamsAs1DForOutWhenUnconnected=off
  rRegenPaddle : Outport  Port=54  VectorParamsAs1DForOutWhenUnconnected=off
  vChassis : Outport  Port=55  VectorParamsAs1DForOutWhenUnconnected=off
  pBrakeMax : Outport  Port=56  VectorParamsAs1DForOutWhenUnconnected=off
  vWheelRL : Outport  Port=57  VectorParamsAs1DForOutWhenUnconnected=off
  vWheelRR : Outport  Port=58  VectorParamsAs1DForOutWhenUnconnected=off
  vWheelFL : Outport  Port=59  VectorParamsAs1DForOutWhenUnconnected=off
  vWheelFR : Outport  Port=60  VectorParamsAs1DForOutWhenUnconnected=off
  BThrottleError : Outport  Port=61  VectorParamsAs1DForOutWhenUnconnected=off
  tThrottleError : Outport  Port=62  VectorParamsAs1DForOutWhenUnconnected=off
  BBrakeError : Outport  Port=63  VectorParamsAs1DForOutWhenUnconnected=off
  tBrakeError : Outport  Port=64  VectorParamsAs1DForOutWhenUnconnected=off
  BBrakeOn : Outport  Port=65  VectorParamsAs1DForOutWhenUnconnected=off
  BPedalOverlap : Outport  Port=66  VectorParamsAs1DForOutWhenUnconnected=off
  BAppsOK : Outport  Port=67  VectorParamsAs1DForOutWhenUnconnected=off
  BRegenOn : Outport  Port=68  VectorParamsAs1DForOutWhenUnconnected=off
  BTVOn : Outport  Port=69  VectorParamsAs1DForOutWhenUnconnected=off
  rSOE : Outport  Port=70  VectorParamsAs1DForOutWhenUnconnected=off
  sChassis : Outport  Port=71  VectorParamsAs1DForOutWhenUnconnected=off
  rSOC : Outport  Port=72  VectorParamsAs1DForOutWhenUnconnected=off
  rTVMultiplier : Outport  Port=73  VectorParamsAs1DForOutWhenUnconnected=off
  PEngineBraking : Outport  Port=74  VectorParamsAs1DForOutWhenUnconnected=off
  NInvState : Outport  Port=75  VectorParamsAs1DForOutWhenUnconnected=off
  rGrip : Outport  Port=76  VectorParamsAs1DForOutWhenUnconnected=off
  rSlipRatioFRActual : Outport  Port=77  VectorParamsAs1DForOutWhenUnconnected=off
  rSlipRatioRLActual : Outport  Port=78  VectorParamsAs1DForOutWhenUnconnected=off
  rSlipRatioRRActual : Outport  Port=79  VectorParamsAs1DForOutWhenUnconnected=off
  NTractionControlMultiplierRR : Outport  Port=80  VectorParamsAs1DForOutWhenUnconnected=off
  NABSMultiplierRR : Outport  Port=81  VectorParamsAs1DForOutWhenUnconnected=off
  NTractionControlMultiplierRL : Outport  Port=82  VectorParamsAs1DForOutWhenUnconnected=off
  NABSMultiplierRL : Outport  Port=83  VectorParamsAs1DForOutWhenUnconnected=off
  NThrottleMap : Outport  Port=84  VectorParamsAs1DForOutWhenUnconnected=off
  BReadyToDrive : Outport  Port=85  VectorParamsAs1DForOutWhenUnconnected=off
  NABSMultiplierFL : Outport  Port=86  VectorParamsAs1DForOutWhenUnconnected=off
  NABSMultiplierFR : Outport  Port=87  VectorParamsAs1DForOutWhenUnconnected=off
  BBalancingOnOut : Outport  Port=88  VectorParamsAs1DForOutWhenUnconnected=off
  MTorqueVectoringFL : Outport  Port=89  VectorParamsAs1DForOutWhenUnconnected=off
  MTorqueVectoringFR : Outport  Port=90  VectorParamsAs1DForOutWhenUnconnected=off
  MTorqueVectoringRL : Outport  Port=91  VectorParamsAs1DForOutWhenUnconnected=off
  MTorqueVectoringRR : Outport  Port=92  VectorParamsAs1DForOutWhenUnconnected=off
  NTractionControlMultiplierFL : Outport  Port=93  VectorParamsAs1DForOutWhenUnconnected=off
  NTractionControlMultiplierFR : Outport  Port=94  VectorParamsAs1DForOutWhenUnconnected=off
  MDischargeLimited : Outport  Port=95  VectorParamsAs1DForOutWhenUnconnected=off
  MDriverRegenRequested : Outport  Port=96  VectorParamsAs1DForOutWhenUnconnected=off
  rSlipRatioOptimal : Outport  Port=97  VectorParamsAs1DForOutWhenUnconnected=off
  NCarState : Outport  Port=98  VectorParamsAs1DForOutWhenUnconnected=off
  MTorqueDistributionFL : Outport  Port=99  VectorParamsAs1DForOutWhenUnconnected=off
  MTorqueDistributionFR : Outport  Port=100  VectorParamsAs1DForOutWhenUnconnected=off
  MTorqueDistributionRL : Outport  Port=101  VectorParamsAs1DForOutWhenUnconnected=off
  MTorqueDistributionRR : Outport  Port=102  VectorParamsAs1DForOutWhenUnconnected=off
  nMotorRLOut : Outport  Port=103  VectorParamsAs1DForOutWhenUnconnected=off
  nMotorFLOut : Outport  Port=104  VectorParamsAs1DForOutWhenUnconnected=off
  nMotorRROut : Outport  Port=105  VectorParamsAs1DForOutWhenUnconnected=off
  nMotorFROut : Outport  Port=106  VectorParamsAs1DForOutWhenUnconnected=off
  BDischargeAllowed : Outport  Port=107  VectorParamsAs1DForOutWhenUnconnected=off
  TMotorRLOut : Outport  Port=108  VectorParamsAs1DForOutWhenUnconnected=off
  TInvRLOut : Outport  Port=109  VectorParamsAs1DForOutWhenUnconnected=off
  TMotorFLOut : Outport  Port=110  VectorParamsAs1DForOutWhenUnconnected=off
  TInvFLOut : Outport  Port=111  VectorParamsAs1DForOutWhenUnconnected=off
  TMotorRROut : Outport  Port=112  VectorParamsAs1DForOutWhenUnconnected=off
  TInvRROut : Outport  Port=113  VectorParamsAs1DForOutWhenUnconnected=off
  TMotorFROut : Outport  Port=114  VectorParamsAs1DForOutWhenUnconnected=off
  TInvFROut : Outport  Port=115  VectorParamsAs1DForOutWhenUnconnected=off
  TInvMax : Outport  Port=116  VectorParamsAs1DForOutWhenUnconnected=off
  TMotorMax : Outport  Port=117  VectorParamsAs1DForOutWhenUnconnected=off
  TCellMaxOut : Outport  Port=118  VectorParamsAs1DForOutWhenUnconnected=off
  IBMSHallEffectOut : Outport  Port=119  VectorParamsAs1DForOutWhenUnconnected=off
  VDCInvRLOut : Outport  Port=120  VectorParamsAs1DForOutWhenUnconnected=off
  BEMSOn : Outport  Port=121  VectorParamsAs1DForOutWhenUnconnected=off
  BTCOn : Outport  Port=122  VectorParamsAs1DForOutWhenUnconnected=off
  VCellMinOut : Outport  Port=123  VectorParamsAs1DForOutWhenUnconnected=off
  VCellMaxOut : Outport  Port=124  VectorParamsAs1DForOutWhenUnconnected=off
  TCellMinOut : Outport  Port=125  VectorParamsAs1DForOutWhenUnconnected=off
  nYawRateErrorActual : Outport  Port=126  VectorParamsAs1DForOutWhenUnconnected=off
  tPedalOverlap : Outport  Port=127  VectorParamsAs1DForOutWhenUnconnected=off
  tAppsTimer : Outport  Port=128  VectorParamsAs1DForOutWhenUnconnected=off
  rSplitRear : Outport  Port=129  VectorParamsAs1DForOutWhenUnconnected=off
  PRegenLimit : Outport  Port=130  VectorParamsAs1DForOutWhenUnconnected=off
  PRegenRequested : Outport  Port=131  VectorParamsAs1DForOutWhenUnconnected=off
  BIMUOk : Outport  Port=132  VectorParamsAs1DForOutWhenUnconnected=off
  EOffset : Outport  Port=133  VectorParamsAs1DForOutWhenUnconnected=off
  PEnergyMeter : Outport  Port=134  VectorParamsAs1DForOutWhenUnconnected=off
  NBMSState : Outport  Port=135  VectorParamsAs1DForOutWhenUnconnected=off
  BOverpower : Outport  Port=136  VectorParamsAs1DForOutWhenUnconnected=off
  BPCComplete : Outport  Port=137  VectorParamsAs1DForOutWhenUnconnected=off
  BEMSDriverSignal1 : Outport  Port=138  VectorParamsAs1DForOutWhenUnconnected=off
  BEMSDriverSignal2 : Outport  Port=139  VectorParamsAs1DForOutWhenUnconnected=off
  BEMSDriverSignal3 : Outport  Port=140  VectorParamsAs1DForOutWhenUnconnected=off
  BPageUp : Outport  Port=141  VectorParamsAs1DForOutWhenUnconnected=off
  BPageDown : Outport  Port=142  VectorParamsAs1DForOutWhenUnconnected=off
  MRegenMax : Outport  Port=143  VectorParamsAs1DForOutWhenUnconnected=off
  NSectorLap : Outport  Port=144  VectorParamsAs1DForOutWhenUnconnected=off
  MPCRegenRequested : Outport  Port=145  VectorParamsAs1DForOutWhenUnconnected=off
  MPCDischargeRequested : Outport  Port=146  VectorParamsAs1DForOutWhenUnconnected=off
  PPCIntegralTermDischarge : Outport  Port=147  VectorParamsAs1DForOutWhenUnconnected=off
  PPCIntegralTermRegen : Outport  Port=148  VectorParamsAs1DForOutWhenUnconnected=off
  NSectorGlobal : Outport  Port=149  VectorParamsAs1DForOutWhenUnconnected=off
  PPCProportionalTermDischarge : Outport  Port=150  VectorParamsAs1DForOutWhenUnconnected=off
  PPCProportionalTermRegen : Outport  Port=151  VectorParamsAs1DForOutWhenUnconnected=off
  BDataMark : Outport  Port=152  VectorParamsAs1DForOutWhenUnconnected=off
  xDamperFL : Outport  Port=153  VectorParamsAs1DForOutWhenUnconnected=off
  xDamperFR : Outport  Port=154  VectorParamsAs1DForOutWhenUnconnected=off
  xDamperRR : Outport  Port=155  VectorParamsAs1DForOutWhenUnconnected=off
  xDamperRL : Outport  Port=156  VectorParamsAs1DForOutWhenUnconnected=off
  BErrorReset : Outport  Port=157  VectorParamsAs1DForOutWhenUnconnected=off
  BDrivetrainCoolingOn : Outport  Port=158  VectorParamsAs1DForOutWhenUnconnected=off
  PPCRegenRequested : Outport  Port=159  VectorParamsAs1DForOutWhenUnconnected=off
  PDischargeLimit : Outport  Port=160  VectorParamsAs1DForOutWhenUnconnected=off
  PRegenDerate : Outport  Port=161  VectorParamsAs1DForOutWhenUnconnected=off
  PHighCellVoltageRegenDerate : Outport  Port=162  VectorParamsAs1DForOutWhenUnconnected=off
  PHighCellTemperatureDerate : Outport  Port=163  VectorParamsAs1DForOutWhenUnconnected=off
  PDischargeDerate : Outport  Port=164  VectorParamsAs1DForOutWhenUnconnected=off
  PMotorTemperatureDerate : Outport  Port=165  VectorParamsAs1DForOutWhenUnconnected=off
  PMotorTemperatureDerateFL : Outport  Port=166  VectorParamsAs1DForOutWhenUnconnected=off
  PMotorTemperatureDerateFR : Outport  Port=167  VectorParamsAs1DForOutWhenUnconnected=off
  PMotorTemperatureDerateRL : Outport  Port=168  VectorParamsAs1DForOutWhenUnconnected=off
  PMotorTemperatureDerateRR : Outport  Port=169  VectorParamsAs1DForOutWhenUnconnected=off
  PLowCellVoltageDischargeDerate : Outport  Port=170  VectorParamsAs1DForOutWhenUnconnected=off
  PInvTemperatureDerate : Outport  Port=171  VectorParamsAs1DForOutWhenUnconnected=off
  PInvTemperatureDerateFL : Outport  Port=172  VectorParamsAs1DForOutWhenUnconnected=off
  PInvTemperatureDerateFR : Outport  Port=173  VectorParamsAs1DForOutWhenUnconnected=off
  PInvTemperatureDerateRR : Outport  Port=174  VectorParamsAs1DForOutWhenUnconnected=off
  PInvTemperatureDerateRL : Outport  Port=175  VectorParamsAs1DForOutWhenUnconnected=off
  aCamberGainSteerFL : Outport  Port=176  VectorParamsAs1DForOutWhenUnconnected=off
  aCamberGainSteerFR : Outport  Port=177  VectorParamsAs1DForOutWhenUnconnected=off
  PPCDischargeRequested : Outport  Port=178  VectorParamsAs1DForOutWhenUnconnected=off
  rSlipRatioFLActual : Outport  Port=179  VectorParamsAs1DForOutWhenUnconnected=off
  FLongitudinalLoadTransfer : Outport  Port=180  VectorParamsAs1DForOutWhenUnconnected=off
  FTyreVerticalFL : Outport  Port=181  VectorParamsAs1DForOutWhenUnconnected=off
  FTyreVerticalFR : Outport  Port=182  VectorParamsAs1DForOutWhenUnconnected=off
  FTyreVerticalRL : Outport  Port=183  VectorParamsAs1DForOutWhenUnconnected=off
  FTyreVerticalRR : Outport  Port=184  VectorParamsAs1DForOutWhenUnconnected=off
  BCalibrationOn : Outport  Port=185  VectorParamsAs1DForOutWhenUnconnected=off
  FTotalDownforce : Outport  Port=186  VectorParamsAs1DForOutWhenUnconnected=off
  aSlipAngleFL : Outport  Port=187  VectorParamsAs1DForOutWhenUnconnected=off
  aSlipAngleFR : Outport  Port=188  VectorParamsAs1DForOutWhenUnconnected=off
  aCamberFL : Outport  Port=189  VectorParamsAs1DForOutWhenUnconnected=off
  aCamberFR : Outport  Port=190  VectorParamsAs1DForOutWhenUnconnected=off
  aCamberRL : Outport  Port=191  VectorParamsAs1DForOutWhenUnconnected=off
  aCamberRR : Outport  Port=192  VectorParamsAs1DForOutWhenUnconnected=off
  aRollAngle : Outport  Port=193  VectorParamsAs1DForOutWhenUnconnected=off
  xHeaveTravelR : Outport  Port=194  VectorParamsAs1DForOutWhenUnconnected=off
  xHeaveTravelF : Outport  Port=195  VectorParamsAs1DForOutWhenUnconnected=off
  rSpeedRegenDerateFR : Outport  Port=196  VectorParamsAs1DForOutWhenUnconnected=off
  rSpeedRegenDerateRL : Outport  Port=197  VectorParamsAs1DForOutWhenUnconnected=off
  rSpeedRegenDerateFL : Outport  Port=198  VectorParamsAs1DForOutWhenUnconnected=off
  PTSTemperatureDerateFL : Outport  Port=199  VectorParamsAs1DForOutWhenUnconnected=off
  PTSTemperatureDerateFR : Outport  Port=200  VectorParamsAs1DForOutWhenUnconnected=off
  PTSTemperatureDerateRL : Outport  Port=201  VectorParamsAs1DForOutWhenUnconnected=off
  PTSTemperatureDerateRR : Outport  Port=202  VectorParamsAs1DForOutWhenUnconnected=off
  PSOCDischargeDerate : Outport  Port=203  VectorParamsAs1DForOutWhenUnconnected=off
  PSOCRegenDerate : Outport  Port=204  VectorParamsAs1DForOutWhenUnconnected=off
  aSlipAngleRL : Outport  Port=205  VectorParamsAs1DForOutWhenUnconnected=off
  aSlipAngleRR : Outport  Port=206  VectorParamsAs1DForOutWhenUnconnected=off
  BSpeedDerateOn : Outport  Port=207  VectorParamsAs1DForOutWhenUnconnected=off
  VDCAccumulatorOut : Outport  Port=208  VectorParamsAs1DForOutWhenUnconnected=off
  MTractionControlRRTotal : Outport  Port=209  VectorParamsAs1DForOutWhenUnconnected=off
  MTractionControlRLTotal : Outport  Port=210  VectorParamsAs1DForOutWhenUnconnected=off
  MTractionControlFRTotal : Outport  Port=211  VectorParamsAs1DForOutWhenUnconnected=off
  MTractionControlFLTotal : Outport  Port=212  VectorParamsAs1DForOutWhenUnconnected=off
  BSpinningModeOn : Outport  Port=213  VectorParamsAs1DForOutWhenUnconnected=off
  PRegenMax : Outport  Port=214  VectorParamsAs1DForOutWhenUnconnected=off
  rEngineBrakingSplit : Outport  Port=215  VectorParamsAs1DForOutWhenUnconnected=off
  NLap : Outport  Port=216  VectorParamsAs1DForOutWhenUnconnected=off
  sSector : Outport  Port=217  VectorParamsAs1DForOutWhenUnconnected=off
  EBudget : Outport  Port=218  VectorParamsAs1DForOutWhenUnconnected=off
  ERemaining : Outport  Port=219  VectorParamsAs1DForOutWhenUnconnected=off
  ESector : Outport  Port=220  VectorParamsAs1DForOutWhenUnconnected=off
  FTotalLateralLoadTransfer : Outport  Port=221  VectorParamsAs1DForOutWhenUnconnected=off
  BAccuFanOn : Outport  Port=222  VectorParamsAs1DForOutWhenUnconnected=off
  BMotorRBHFanOn : Outport  Port=223  VectorParamsAs1DForOutWhenUnconnected=off
  BInverterFanOn : Outport  Port=224  VectorParamsAs1DForOutWhenUnconnected=off
  BReadyToDriveBuzzer : Outport  Port=225  VectorParamsAs1DForOutWhenUnconnected=off
  BBrakeLight : Outport  Port=226  VectorParamsAs1DForOutWhenUnconnected=off
  BInvLVOn : Outport  Port=227  VectorParamsAs1DForOutWhenUnconnected=off
  tIMUError : Outport  Port=228  VectorParamsAs1DForOutWhenUnconnected=off
  MDriverDischargeRequested : Outport  Port=229  VectorParamsAs1DForOutWhenUnconnected=off
  MRegenLimited : Outport  Port=230  VectorParamsAs1DForOutWhenUnconnected=off
  MTotalRequested : Outport  Port=231  VectorParamsAs1DForOutWhenUnconnected=off
  BxDamperFLOk : Outport  Port=232  VectorParamsAs1DForOutWhenUnconnected=off
  BxDamperFROk : Outport  Port=233  VectorParamsAs1DForOutWhenUnconnected=off
  BxDamperRLOk : Outport  Port=234  VectorParamsAs1DForOutWhenUnconnected=off
  BxDamperRROk : Outport  Port=235  VectorParamsAs1DForOutWhenUnconnected=off
  BIMUError : Outport  Port=236  VectorParamsAs1DForOutWhenUnconnected=off
  PDischargeLimited : Outport  Port=237  VectorParamsAs1DForOutWhenUnconnected=off
  aCamberGainRollF : Outport  Port=238  VectorParamsAs1DForOutWhenUnconnected=off
  aCamberGainRollR : Outport  Port=239  VectorParamsAs1DForOutWhenUnconnected=off
  aCamberGainHeaveF : Outport  Port=240  VectorParamsAs1DForOutWhenUnconnected=off
  aCamberGainHeaveR : Outport  Port=241  VectorParamsAs1DForOutWhenUnconnected=off
  BInverterErrorRear : Outport  Port=242  VectorParamsAs1DForOutWhenUnconnected=off
  BInverterErrorFront : Outport  Port=243  VectorParamsAs1DForOutWhenUnconnected=off
  ETotalRequested : Outport  Port=244  VectorParamsAs1DForOutWhenUnconnected=off
  ESector1Remaining : Outport  Port=245  VectorParamsAs1DForOutWhenUnconnected=off
  ESector2Remaining : Outport  Port=246  VectorParamsAs1DForOutWhenUnconnected=off
  ESector3Remaining : Outport  Port=247  VectorParamsAs1DForOutWhenUnconnected=off
  ESector4Remaining : Outport  Port=248  VectorParamsAs1DForOutWhenUnconnected=off
  NSector9Remaining : Outport  Port=249  VectorParamsAs1DForOutWhenUnconnected=off
  NSector10Remaining : Outport  Port=250  VectorParamsAs1DForOutWhenUnconnected=off
  NSector11Remaining : Outport  Port=251  VectorParamsAs1DForOutWhenUnconnected=off
  NSector12Remaining : Outport  Port=252  VectorParamsAs1DForOutWhenUnconnected=off
  ESector5Remaining : Outport  Port=253  VectorParamsAs1DForOutWhenUnconnected=off
  ESector6Remaining : Outport  Port=254  VectorParamsAs1DForOutWhenUnconnected=off
  ESector7Remaining : Outport  Port=255  VectorParamsAs1DForOutWhenUnconnected=off
  ESector9Remaining : Outport  Port=256  VectorParamsAs1DForOutWhenUnconnected=off
  ESector10Remaining : Outport  Port=257  VectorParamsAs1DForOutWhenUnconnected=off
  ESector11Remaining : Outport  Port=258  VectorParamsAs1DForOutWhenUnconnected=off
  ESector12Remaining : Outport  Port=259  VectorParamsAs1DForOutWhenUnconnected=off
  NSector1Remaining : Outport  Port=260  VectorParamsAs1DForOutWhenUnconnected=off
  NSector2Remaining : Outport  Port=261  VectorParamsAs1DForOutWhenUnconnected=off
  NSector3Remaining : Outport  Port=262  VectorParamsAs1DForOutWhenUnconnected=off
  NSector4Remaining : Outport  Port=263  VectorParamsAs1DForOutWhenUnconnected=off
  NSector5Remaining : Outport  Port=264  VectorParamsAs1DForOutWhenUnconnected=off
  NSector6Remaining : Outport  Port=265  VectorParamsAs1DForOutWhenUnconnected=off
  NSector7Remaining : Outport  Port=266  VectorParamsAs1DForOutWhenUnconnected=off
  NSector8Remaining : Outport  Port=267  VectorParamsAs1DForOutWhenUnconnected=off
  ESector8Remaining : Outport  Port=268  VectorParamsAs1DForOutWhenUnconnected=off
  NThrottleMapEM : Outport  Port=269  VectorParamsAs1DForOutWhenUnconnected=off
  NThrottleMapOW : Outport  Port=270  VectorParamsAs1DForOutWhenUnconnected=off
  rTorqueSplit : Outport  Port=271  VectorParamsAs1DForOutWhenUnconnected=off
  rTorqueSplitOW : Outport  Port=272  VectorParamsAs1DForOutWhenUnconnected=off
  PRegenMaxEM : Outport  Port=273  VectorParamsAs1DForOutWhenUnconnected=off
  PRegenMaxOW : Outport  Port=274  VectorParamsAs1DForOutWhenUnconnected=off
  rTVMultiplierEM : Outport  Port=275  VectorParamsAs1DForOutWhenUnconnected=off
  rTVMultiplierOW : Outport  Port=276  VectorParamsAs1DForOutWhenUnconnected=off
  rEngineBrakingSplitEM : Outport  Port=277  VectorParamsAs1DForOutWhenUnconnected=off
  rEngineBrakingSplitOW : Outport  Port=278  VectorParamsAs1DForOutWhenUnconnected=off
  PDischargeMaxEM : Outport  Port=279  VectorParamsAs1DForOutWhenUnconnected=off
  PDischargeMaxOW : Outport  Port=280  VectorParamsAs1DForOutWhenUnconnected=off
  PEngineBrakingEM : Outport  Port=281  VectorParamsAs1DForOutWhenUnconnected=off
  PEngineBrakingOW : Outport  Port=282  VectorParamsAs1DForOutWhenUnconnected=off
  NTCKdSelector : Outport  Port=283  VectorParamsAs1DForOutWhenUnconnected=off
  NPCKpSelector : Outport  Port=284  VectorParamsAs1DForOutWhenUnconnected=off
  rTorqueSplitEM : Outport  Port=285  VectorParamsAs1DForOutWhenUnconnected=off
  BTVOnEM : Outport  Port=286  VectorParamsAs1DForOutWhenUnconnected=off
  BTVOnOW : Outport  Port=287  VectorParamsAs1DForOutWhenUnconnected=off
  BDrivetrainCoolingOnEM : Outport  Port=288  VectorParamsAs1DForOutWhenUnconnected=off
  BDrivetrainCoolingOnOW : Outport  Port=289  VectorParamsAs1DForOutWhenUnconnected=off
  BTCOnEM : Outport  Port=290  VectorParamsAs1DForOutWhenUnconnected=off
  BTCOnOW : Outport  Port=291  VectorParamsAs1DForOutWhenUnconnected=off
  BEMSOnEM : Outport  Port=292  VectorParamsAs1DForOutWhenUnconnected=off
  BEMSOnOW : Outport  Port=293  VectorParamsAs1DForOutWhenUnconnected=off
  BSpinningModeOnEM : Outport  Port=294  VectorParamsAs1DForOutWhenUnconnected=off
  BSpinningModeOnOW : Outport  Port=295  VectorParamsAs1DForOutWhenUnconnected=off
  NEventMode : Outport  Port=296  VectorParamsAs1DForOutWhenUnconnected=off
  BInvErrorResetRLCAN3 : Outport  Port=297  VectorParamsAs1DForOutWhenUnconnected=off
  BInvErrorResetFLCAN3 : Outport  Port=298  VectorParamsAs1DForOutWhenUnconnected=off
  BInvErrorResetFRCAN3 : Outport  Port=299  VectorParamsAs1DForOutWhenUnconnected=off
  BInvErrorResetRRCAN3 : Outport  Port=300  VectorParamsAs1DForOutWhenUnconnected=off
  BQuitInvOnFLCAN3 : Outport  Port=301  VectorParamsAs1DForOutWhenUnconnected=off
  BQuitInvOnFRCAN3 : Outport  Port=302  VectorParamsAs1DForOutWhenUnconnected=off
  BQuitInvOnRRCAN3 : Outport  Port=303  VectorParamsAs1DForOutWhenUnconnected=off
  BQuitInvOnRLCAN3 : Outport  Port=304  VectorParamsAs1DForOutWhenUnconnected=off
  wires:
  nMotorRL/1 -> Bus Creator17/1  "nMotorRL"
  BInvDCOnRLIn/1 -> Bus Creator17/2  "BInvDCOnRLIn"
  BInvErrorRL/1 -> Bus Creator17/3  "BInvErrorRL"
  BInvOnRLIn/1 -> Bus Creator17/4  "BInvOnRLIn"
  BInvQuitDcOnRL/1 -> Bus Creator17/5  "BInvQuitDcOnRL"
  BInvSysReadyRL/1 -> Bus Creator17/7  "BInvSysReadyRL"
  BInvWarnRL/1 -> Bus Creator17/8  "BInvWarnRL"
  MMotorMeasuredRL/1 -> Bus Creator17/9  "MMotorMeasuredRL"
  NInvDTCRL/1 -> Bus Creator17/10  "NInvDTCRL"
  TMotorRL/1 -> Bus Creator17/11  "TMotorRL"
  VDCInvRL/1 -> Bus Creator17/12  "VDCInvRL"
  MMotorMeasuredRR/1 -> Bus Creator19/9  "MMotorMeasuredRR"
  BInvSysReadyRR/1 -> Bus Creator19/7  "BInvSysReadyRR"
  TMotorRR/1 -> Bus Creator19/11  "TMotorRR"
  BInvErrorRR/1 -> Bus Creator19/3  "BInvErrorRR"
  nMotorRR/1 -> Bus Creator19/1  "nMotorRR"
  BInvQuitDcOnRR/1 -> Bus Creator19/5  "BInvQuitDcOnRR"
  BInvDCOnRRIn/1 -> Bus Creator19/2  "BInvDCOnRRIn"
  BInvWarnRR/1 -> Bus Creator19/8  "BInvWarnRR"
  NInvDTCRR/1 -> Bus Creator19/10  "NInvDTCRR"
  VDCInvRR/1 -> Bus Creator19/12  "VDCInvRR"
  BInvOnRRIn/1 -> Bus Creator19/4  "BInvOnRRIn"
  BInvOnFLIn/1 -> Bus Creator14/4  "BInvOnFLIn"
  VDCInvFL/1 -> Bus Creator14/12  "VDCInvFL"
  BInvWarnFL/1 -> Bus Creator14/8  "BInvWarnFL"
  BInvQuitDcOnFL/1 -> Bus Creator14/5  "BInvQuitDcOnFL"
  NInvDTCFL/1 -> Bus Creator14/10  "NInvDTCFL"
  BInvErrorFL/1 -> Bus Creator14/3  "BInvErrorFL"
  BInvDCOnFLIn/1 -> Bus Creator14/2  "BInvDCOnFLIn"
  TMotorFL/1 -> Bus Creator14/11  "TMotorFL"
  nMotorFL/1 -> Bus Creator14/1  "nMotorFL"
  BInvSysReadyFL/1 -> Bus Creator14/7  "BInvSysReadyFL"
  MMotorMeasuredFL/1 -> Bus Creator14/9  "MMotorMeasuredFL"
  BInvDCOnFRIn/1 -> Bus Creator15/2  "BInvDCOnFRIn"
  BInvErrorFR/1 -> Bus Creator15/3  "BInvErrorFR"
  MMotorMeasuredFR/1 -> Bus Creator15/9  "MMotorMeasuredFR"
  BInvSysReadyFR/1 -> Bus Creator15/7  "BInvSysReadyFR"
  nMotorFR/1 -> Bus Creator15/1  "nMotorFR"
  TMotorFR/1 -> Bus Creator15/11  "TMotorFR"
  NInvDTCFR/1 -> Bus Creator15/10  "NInvDTCFR"
  VDCInvFR/1 -> Bus Creator15/12  "VDCInvFR"
  BInvQuitDcOnFR/1 -> Bus Creator15/5  "BInvQuitDcOnFR"
  BInvWarnFR/1 -> Bus Creator15/8  "BInvWarnFR"
  BInvOnFRIn/1 -> Bus Creator15/4  "BInvOnFRIn"
  Bus Creator17/1 -> [InverterRL]
  Bus Creator14/1 -> [InverterFL]
  Bus Creator15/1 -> [InverterFR]
  IIVTS/1 -> Bus Creator18/1  "IIVTS"
  TCellMin/1 -> Bus Creator18/4  "TCellMin"
  RCellAverage/1 -> Bus Creator18/10  "RCellAverage"
  TCellMax/1 -> Bus Creator18/7  "TCellMax"
  BBMSP0A80/1 -> Bus Creator18/15  "BBMSP0A80"
  IBMSHallEffect/1 -> Bus Creator18/2  "IBMSHallEffect"
  VDCAccumulator/1 -> Bus Creator18/3  "VDCAccumulator"
  VCellAverage/1 -> Bus Creator18/5  "VCellAverage"
  IBMSDCL/1 -> Bus Creator18/8  "IBMSDCL"
  VCellMin/1 -> Bus Creator18/9  "VCellMin"
  VCellMax/1 -> Bus Creator18/6  "VCellMax"
  BBalancingOn/1 -> Bus Creator18/11  "BBalancingOn"
  BBMSP0A0C/1 -> Bus Creator18/12  "BBMSP0A0C"
  BBMSP0A0E/1 -> Bus Creator18/13  "BBMSP0A0E"
  BBMSP0A10/1 -> Bus Creator18/14  "BBMSP0A10"
  BBMSP0AC0/1 -> Bus Creator18/16  "BBMSP0AC0"
  BBMSP0AFA/1 -> Bus Creator18/17  "BBMSP0AFA"
  Bus Creator18/1 -> [BMS]
  CAN1_2Bus/1 -> Model/1
  [BMS] -> Model/3
  Bus Creator/1 -> Model/2
  Model/1 -> [Global]
  TInvRL/1 -> Bus Creator17/13  "TInvRL"
  TInvRR/1 -> Bus Creator19/13  "TInvRR"
  TInvFL/1 -> Bus Creator14/13  "TInvFL"
  TInvFR/1 -> Bus Creator15/13  "TInvFR"
  BQuitInvOnRL/1 -> Bus Creator17/6  "BQuitInvOnRL"
  BQuitInvOnRR/1 -> Bus Creator19/6  "BQuitInvOnRR"
  BQuitInvOnFL/1 -> Bus Creator14/6  "BQuitInvOnFL"
  BQuitInvOnFR/1 -> Bus Creator15/6  "BQuitInvOnFR"
  [Global] -> Bus Selector1/1
  [Global] -> Bus Selector2/1
  [Global] -> Bus Selector3/1
  [Global] -> Bus Selector4/1
  [Global] -> Bus Selector6/1
  [Global] -> Bus Selector7/1
  [Global] -> Bus Selector8/1
  [Global] -> Bus Selector9/1
  [Global] -> Bus Selector10/1
  [Global] -> Bus Selector12/1
  [Global] -> Bus Selector13/1
  [Global] -> Bus Selector14/1
  [Global] -> Bus Selector15/1
  [Global] -> Bus Selector18/1
  [Global] -> Bus Selector20/1
  Bus Selector20/1 -> BInvDCOnRLOut/1  "<BInvDCOnRLOut>"
  Bus Selector20/2 -> BInvEnableRL/1  "<BInvEnableRL>"
  Bus Selector20/3 -> BInvErrorResetRL/1  "<BInvErrorResetRL>"
  Bus Selector20/4 -> BInvOnRLOut/1  "<BInvOnRLOut>"
  Bus Selector20/5 -> MTorqueLimitNegativeRL/1  "<MTorqueLimitNegativeRL>"
  Bus Selector20/6 -> MTorqueLimitPositiveRL/1  "<MTorqueLimitPositiveRL>"
  Bus Selector20/7 -> MInvRLFinal/1  "<MRLFinal>"
  [Global] -> Bus Selector21/1
  Bus Selector21/5 -> MTorqueLimitNegativeFL/1  "<MTorqueLimitNegativeFL>"
  Bus Selector21/2 -> BInvEnableFL/1  "<BInvEnableFL>"
  Bus Selector21/7 -> MInvFLFinal/1  "<MFLFinal>"
  Bus Selector21/6 -> MTorqueLimitPositiveFL/1  "<MTorqueLimitPositiveFL>"
  Bus Selector21/3 -> BInvErrorResetFL/1  "<BInvErrorResetFL>"
  Bus Selector21/1 -> BInvDCOnFLOut/1  "<BInvDCOnFLOut>"
  Bus Selector21/4 -> BInvOnFLOut/1  "<BInvOnFLOut>"
  Bus Selector22/4 -> BInvOnRROut/1  "<BInvOnRROut>"
  Bus Selector22/6 -> MTorqueLimitPositiveRR/1  "<MTorqueLimitPositiveRR>"
  Bus Selector22/7 -> MInvRRFinal/1  "<MRRFinal>"
  Bus Selector22/3 -> BInvErrorResetRR/1  "<BInvErrorResetRR>"
  Bus Selector22/1 -> BInvDCOnRROut/1  "<BInvDCOnRROut>"
  [Global] -> Bus Selector22/1
  Bus Selector22/2 -> BInvEnableRR/1  "<BInvEnableRR>"
  Bus Selector22/5 -> MTorqueLimitNegativeRR/1  "<MTorqueLimitNegativeRR>"
  Bus Selector23/2 -> BInvEnableFR/1  "<BInvEnableFR>"
  Bus Selector23/5 -> MTorqueLimitNegativeFR/1  "<MTorqueLimitNegativeFR>"
  Bus Selector23/1 -> BInvDCOnFROut/1  "<BInvDCOnFROut>"
  [Global] -> Bus Selector23/1
  Bus Selector23/3 -> BInvErrorResetFR/1  "<BInvErrorResetFR>"
  Bus Selector23/6 -> MTorqueLimitPositiveFR/1  "<MTorqueLimitPositiveFR>"
  Bus Selector23/4 -> BInvOnFROut/1  "<BInvOnFROut>"
  [InverterRR] -> CAN1_2Bus/4  "InverterRR"
  [InverterRL] -> CAN1_2Bus/3  "InverterRL"
  [InverterFR] -> CAN1_2Bus/2  "InverterFR"
  [InverterFL] -> CAN1_2Bus/1  "InverterFL"
  Bus Creator19/1 -> [InverterRR]
  [Global] -> Bus Selector19/1
  [Global] -> Bus Selector24/1
  [Global] -> Bus Selector29/1
  [Global] -> Bus Selector30/1
  [Global] -> Bus Selector31/1
  [Global] -> Bus Selector33/1
  [Global] -> Bus Selector34/1
  [Global] -> Bus Selector35/1
  [Global] -> Bus Selector42/1
  [Global] -> Bus Selector47/1
  [Global] -> Bus Selector48/1
  [Global] -> Bus Selector49/1
  [Global] -> Bus Selector53/1
  [Global] -> Bus Selector54/1
  [Global] -> Bus Selector38/1
  [Global] -> Bus Selector55/1
  Bus Selector23/7 -> MInvFRFinal/1  "<MFRFinal>"
  [DDU7] -> Bus Creator/2  "DDU7"
  [IMU] -> Bus Creator/3  "IMU"
  [STW] -> Bus Creator/1  "STW"
  [Global] -> Bus Selector/1
  Bus Selector/1 -> MFLFinal/1  "<MFLFinal>"
  Bus Selector/2 -> MFRFinal/1  "<MFRFinal>"
  Bus Selector/3 -> MRLFinal/1  "<MRLFinal>"
  Bus Selector/4 -> MRRFinal/1  "<MRRFinal>"
  Bus Selector/5 -> IIVTSOut/1  "<IIVTS>"
  Bus Selector/6 -> PActual/1  "<PActual>"
  Bus Selector/7 -> BBrakeError/1  "<BBrakeError>"
  Bus Selector/8 -> BThrottleError/1  "<BThrottleError>"
  Bus Selector/9 -> BOverpower/1  "<BOverpower>"
  Bus Selector/10 -> BDischargeAllowed/1  "<BDischargeAllowed>"
  Bus Selector1/1 -> vChassis/1  "<vChassis>"
  Bus Selector1/2 -> PEnergyMeter/1  "<PEnergyMeter>"
  Bus Selector2/1 -> vWheelFL/1  "<vWheelFL>"
  Bus Selector2/2 -> vWheelFR/1  "<vWheelFR>"
  Bus Selector2/3 -> nMotorFLOut/1  "<nMotorFL>"
  Bus Selector2/4 -> nMotorFROut/1  "<nMotorFR>"
  Bus Selector2/5 -> rThrottlePedal1/1  "<rThrottlePedal1>"
  Bus Selector2/6 -> BPageUp/1  "<BPageUp>"
  Bus Selector3/1 -> vWheelRL/1  "<vWheelRL>"
  Bus Selector3/2 -> vWheelRR/1  "<vWheelRR>"
  Bus Selector3/3 -> nMotorRLOut/1  "<nMotorRL>"
  Bus Selector3/4 -> nMotorRROut/1  "<nMotorRR>"
  Bus Selector3/5 -> rThrottlePedal/1  "<rThrottlePedal>"
  Bus Selector3/6 -> BPageDown/1  "<BPageDown>"
  [Global] -> Bus Selector5/1
  Bus Selector5/2 -> rRegenPaddle/1  "<rRegenPaddle>"
  Bus Selector5/1 -> pBrakeMax/1  "<pBrakeMax>"
  Bus Selector5/3 -> xDamperFL/1  "<xDamperFL>"
  Bus Selector5/4 -> xDamperFR/1  "<xDamperFR>"
  Bus Selector5/5 -> xDamperRL/1  "<xDamperRL>"
  Bus Selector5/6 -> xDamperRR/1  "<xDamperRR>"
  Bus Selector5/7 -> BIMUOk/1  "<BIMUOK>"
  Bus Selector5/8 -> tIMUError/1  "<tIMUError>"
  Bus Selector5/9 -> BDataMark/1  "<BDataMark>"
  Bus Selector12/1 -> aSteeringAngle/1  "<aSteeringAngle>"
  Bus Selector12/2 -> PLowCellVoltageDischargeDerate/1  "<PLowCellVoltageDischargeDerate>"
  Bus Selector12/3 -> PHighCellVoltageRegenDerate/1  "<PHighCellVoltageRegenDerate>"
  Bus Selector12/4 -> MDriverDischargeRequested/1  "<MDriverDischargeRequested>"
  Bus Selector12/5 -> MDriverRegenRequested/1  "<MDriverRegenRequested>"
  Bus Selector12/6 -> PPCIntegralTermDischarge/1  "<PPCIntegralTermDischarge>"
  Bus Selector12/7 -> PPCIntegralTermRegen/1  "<PPCIntegralTermRegen>"
  Bus Selector9/1 -> MTorqueVectoringFL/1  "<MTorqueVectoringFL>"
  Bus Selector9/2 -> MTorqueVectoringFR/1  "<MTorqueVectoringFR>"
  Bus Selector9/3 -> MTorqueVectoringRL/1  "<MTorqueVectoringRL>"
  Bus Selector9/4 -> MTorqueVectoringRR/1  "<MTorqueVectoringRR>"
  Bus Selector9/5 -> MTorqueDistributionFL/1  "<MTorqueDistributionFL>"
  Bus Selector9/6 -> MTorqueDistributionFR/1  "<MTorqueDistributionFR>"
  Bus Selector9/7 -> MRegenLimited/1  "<MRegenLimited>"
  Bus Selector4/1 -> tPedalOverlap/1  "<tPedalOverlap>"
  Bus Selector4/2 -> PPCProportionalTermDischarge/1  "<PPCProportionalTermDischarge>"
  Bus Selector4/3 -> MPCDischargeRequested/1  "<MPCDischargeRequested>"
  Bus Selector4/4 -> PPCProportionalTermRegen/1  "<PPCProportionalTermRegen>"
  Bus Selector4/5 -> MPCRegenRequested/1  "<MPCRegenRequested>"
  Bus Selector4/6 -> MDischargeLimited/1  "<MDischargeLimited>"
  Bus Selector4/7 -> NTractionControlMultiplierFL/1  "<NTractionControlMultiplierFL>"
  Bus Selector4/8 -> NTractionControlMultiplierFR/1  "<NTractionControlMultiplierFR>"
  Bus Selector19/1 -> tThrottleError/1  "<tThrottleError>"
  Bus Selector19/2 -> MTorqueDistributionRR/1  "<MTorqueDistributionRR>"
  Bus Selector19/3 -> NTractionControlMultiplierRL/1  "<NTractionControlMultiplierRL>"
  Bus Selector19/4 -> NTractionControlMultiplierRR/1  "<NTractionControlMultiplierRR>"
  Bus Selector19/5 -> NABSMultiplierFL/1  "<NABSMultiplierFL>"
  Bus Selector19/6 -> NABSMultiplierFR/1  "<NABSMultiplierFR>"
  Bus Selector19/7 -> NABSMultiplierRL/1  "<NABSMultiplierRL>"
  Bus Selector19/8 -> FTyreVerticalFL/1  "<FTyreVerticalFL>"
  Bus Selector24/7 -> rSlipRatioRRActual/1  "<rSlipRatioRRActual>"
  Bus Selector24/1 -> tBrakeError/1  "<tBrakeError>"
  Bus Selector24/2 -> nYawRateErrorActual/1  "<nYawRateErrorActual>"
  Bus Selector24/3 -> MTorqueDistributionRL/1  "<MTorqueDistributionRL>"
  Bus Selector24/5 -> MTractionControlFRTotal/1  "<MTractionControlFRTotal>"
  Bus Selector15/1 -> NABSMultiplierRR/1  "<NABSMultiplierRR>"
  Bus Selector15/2 -> MTractionControlRRTotal/1  "<MTractionControlRRTotal>"
  Bus Selector15/3 -> MTotalFinal/1  "<MTotalFinal>"
  Bus Selector15/4 -> rSlipRatioFLActual/1  "<rSlipRatioFLActual>"
  Bus Selector15/5 -> rSlipRatioFRActual/1  "<rSlipRatioFRActual>"
  Bus Selector15/6 -> rSlipRatioRLActual/1  "<rSlipRatioRLActual>"
  Bus Selector15/7 -> FTyreVerticalFR/1  "<FTyreVerticalFR>"
  Bus Selector6/6 -> aSlipAngleRR/1  "<aSlipAngleRR>"
  Bus Selector6/5 -> aSlipAngleRL/1  "<aSlipAngleRL>"
  Bus Selector6/4 -> aSlipAngleFR/1  "<aSlipAngleFR>"
  Bus Selector6/3 -> aSlipAngleFL/1  "<aSlipAngleFL>"
  Bus Selector6/2 -> FTyreVerticalRR/1  "<FTyreVerticalRR>"
  Bus Selector6/1 -> FTyreVerticalRL/1  "<FTyreVerticalRL>"
  Bus Selector29/1 -> NCarState/1  "<NCarState>"
  Bus Selector29/2 -> pBrakeF/1  "<pBrakeF>"
  Bus Selector29/3 -> pBrakeR/1  "<pBrakeR>"
  Bus Selector29/4 -> tAppsTimer/1  "<tAppsTimer>"
  Bus Selector29/5 -> VCellMaxOut/1  "<VCellMax>"
  Bus Selector29/6 -> VCellMinOut/1  "<VCellMin>"
  Bus Selector29/7 -> PSOCDischargeDerate/1  "<PSOCDischargeDerate>"
  Bus Selector30/1 -> rSpeedRegenDerateRL/1  "<rSpeedRegenDerateRL>"
  Bus Selector30/2 -> rSpeedRegenDerateFR/1  "<rSpeedRegenDerateFR>"
  Bus Selector30/3 -> rSpeedRegenDerateFL/1  "<rSpeedRegenDerateFL>"
  Bus Selector30/4 -> BSpeedDerateOn/1  "<BSpeedDerateOn>"
  Bus Selector30/5 -> PDischargeDerate/1  "<PDischargeDerate>"
  Bus Selector30/6 -> PRegenDerate/1  "<PRegenDerate>"
  Bus Selector30/7 -> PRegenRequested/1  "<PRegenRequested>"
  Bus Selector30/8 -> PDischargeLimit/1  "<PDischargeLimit>"
  Bus Selector30/9 -> PRegenLimit/1  "<PRegenLimit>"
  Bus Selector30/10 -> PPCDischargeRequested/1  "<PPCDischargeRequested>"
  Bus Selector10/1 -> MTotalRequested/1  "<MTotalRequested>"
  Bus Selector10/2 -> rSlipRatioOptimal/1  "<rSlipRatioOptimal>"
  Bus Selector10/3 -> aCamberFL/1  "<aCamberFL>"
  Bus Selector10/4 -> aCamberFR/1  "<aCamberFR>"
  Bus Selector10/5 -> aCamberRL/1  "<aCamberRL>"
  Bus Selector10/6 -> aCamberRR/1  "<aCamberRR>"
  Bus Selector10/7 -> FTotalLateralLoadTransfer/1  "<FTotalLateralLoadTransfer>"
  Bus Selector8/1 -> BBrakeOn/1  "<BBrakeOn>"
  Bus Selector8/2 -> BPedalOverlap/1  "<BPedalOverlap>"
  Bus Selector8/3 -> BAppsOK/1  "<BAppsOK>"
  Bus Selector8/4 -> BRegenOn/1  "<BRegenOn>"
  Bus Selector8/5 -> BxDamperFLOk/1  "<BxDamperFLOk>"
  Bus Selector8/6 -> BxDamperFROk/1  "<BxDamperFROk>"
  Bus Selector8/7 -> BxDamperRLOk/1  "<BxDamperRLOk>"
  Bus Selector8/8 -> BxDamperRROk/1  "<BxDamperRROk>"
  Bus Selector8/9 -> BIMUError/1  "<BIMUError>"
  Bus Selector8/10 -> BCalibrationOn/1  "<BCalibrationOn>"
  Bus Selector8/11 -> PSOCRegenDerate/1  "<PSOCRegenDerate>"
  Bus Selector8/12 -> rSpeedRegenDerateRR/1  "<rSpeedRegenDerateRR>"
  Bus Selector8/13 -> PPCRegenRequested/1  "<PPCRegenRequested>"
  Bus Selector8/15 -> BEMSDriverSignal1/1  "<BEMSDriverSignal1>"
  Bus Selector8/16 -> BEMSDriverSignal2/1  "<BEMSDriverSignal2>"
  Bus Selector8/17 -> BEMSDriverSignal3/1  "<BEMSDriverSignal3>"
  Bus Selector8/18 -> FLongitudinalLoadTransfer/1  "<FLongitudinalLoadTransfer>"
  Bus Selector14/1 -> sChassis/1  "<sChassis>"
  Bus Selector14/2 -> PInvTemperatureDerate/1  "<PInvTemperatureDerate>"
  Bus Selector14/3 -> PInvTemperatureDerateFR/1  "<PInvTemperatureDerateFR>"
  Bus Selector14/4 -> PInvTemperatureDerateFL/1  "<PInvTemperatureDerateFL>"
  Bus Selector14/5 -> PInvTemperatureDerateRR/1  "<PInvTemperatureDerateRR>"
  Bus Selector14/6 -> IBMSHallEffectOut/1  "<IBMSHallEffect>"
  Bus Selector8/14 -> PDischargeLimited/1  "<PDischargeLimited>"
  Bus Selector42/1 -> PInvTemperatureDerateRL/1  "<PInvTemperatureDerateRL>"
  Bus Selector42/2 -> PMotorTemperatureDerate/1  "<PMotorTemperatureDerate>"
  Bus Selector42/3 -> PMotorTemperatureDerateFR/1  "<PMotorTemperatureDerateFR>"
  Bus Selector42/4 -> PMotorTemperatureDerateFL/1  "<PMotorTemperatureDerateFL>"
  Bus Selector42/5 -> PMotorTemperatureDerateRR/1  "<PMotorTemperatureDerateRR>"
  Bus Selector42/6 -> aCamberGainSteerFL/1  "<aCamberGainSteerFL>"
  Bus Selector42/7 -> aCamberGainSteerFR/1  "<aCamberGainSteerFR>"
  Bus Selector35/1 -> ERemaining/1  "<ERemaining>"
  Bus Selector35/2 -> FTotalDownforce/1  "<FTotalDownforce>"
  Bus Selector35/3 -> aCamberGainRollF/1  "<aCamberGainRollF>"
  Bus Selector35/4 -> aCamberGainRollR/1  "<aCamberGainRollR>"
  Bus Selector35/5 -> aCamberGainHeaveF/1  "<aCamberGainHeaveF>"
  Bus Selector35/6 -> aCamberGainHeaveR/1  "<aCamberGainHeaveR>"
  Bus Selector35/7 -> aRollAngle/1  "<aRollAngle>"
  Bus Selector47/1 -> PMotorTemperatureDerateRL/1  "<PMotorTemperatureDerateRL>"
  Bus Selector47/2 -> PTSTemperatureDerateFR/1  "<PTSTemperatureDerateFR>"
  Bus Selector47/3 -> PTSTemperatureDerateFL/1  "<PTSTemperatureDerateFL>"
  Bus Selector47/6 -> PHighCellTemperatureDerate/1  "<PHighCellTemperatureDerate>"
  Bus Selector47/5 -> PTSTemperatureDerateRL/1  "<PTSTemperatureDerateRL>"
  Bus Selector47/4 -> PTSTemperatureDerateRR/1  "<PTSTemperatureDerateRR>"
  Bus Selector48/1 -> ESector/1  "<ESector>"
  Bus Selector48/2 -> xHeaveTravelF/1  "<xHeaveTravelF>"
  Bus Selector48/3 -> xHeaveTravelR/1  "<xHeaveTravelR>"
  Bus Selector31/1 -> BPCComplete/1  "<BPCComplete>"
  Bus Selector31/2 -> BBrakeLight/1  "<BBrakeLight>"
  Bus Selector31/3 -> BReadyToDriveBuzzer/1  "<BReadyToDriveBuzzer>"
  Bus Selector31/4 -> BAccuFanOn/1  "<BAccuFanOn>"
  Bus Selector31/5 -> BMotorRBHFanOn/1  "<BMotorRBHFanOn>"
  Bus Selector31/6 -> BInverterFanOn/1  "<BInverterFanOn>"
  Bus Selector31/7 -> BInvLVOn/1  "<BInvLVOn>"
  Bus Selector33/1 -> TMotorMax/1  "<TMotorMax>"
  Bus Selector33/2 -> TInvMax/1  "<TInvMax>"
  Bus Selector33/3 -> TMotorRLOut/1  "<TMotorRL>"
  Bus Selector33/4 -> VDCInvRLOut/1  "<VDCInvRL>"
  Bus Selector33/5 -> TMotorRROut/1  "<TMotorRR>"
  Bus Selector33/6 -> TMotorFLOut/1  "<TMotorFL>"
  Bus Selector49/1 -> NBMSState/1  "<NBMSState>"
  Bus Selector49/2 -> TInvRROut/1  "<TInvRR>"
  Bus Selector49/7 -> rSplitRear/1  "<rSplitRear>"
  Bus Selector49/6 -> TCellMinOut/1  "<TCellMin>"
  Bus Selector49/5 -> TCellMaxOut/1  "<TCellMax>"
  Bus Selector49/4 -> TInvFROut/1  "<TInvFR>"
  Bus Selector49/3 -> TInvFLOut/1  "<TInvFL>"
  Bus Selector13/1 -> NInvState/1  "<NInvState>"
  Bus Selector13/2 -> BInverterErrorRear/1  "<BInverterErrorRear>"
  Bus Selector13/3 -> BInverterErrorFront/1  "<BInverterErrorFront>"
  Bus Selector13/4 -> BErrorReset/1  "<BErrorReset>"
  Bus Selector13/5 -> TInvRLOut/1  "<TInvRL>"
  Bus Selector13/6 -> TMotorFROut/1  "<TMotorFR>"
  Bus Selector13/7 -> VDCAccumulatorOut/1  "<VDCAccumulator>"
  Bus Selector13/8 -> EBudget/1  "<EBudget>"
  Bus Selector13/9 -> BTVOK/1  "<BTVOK>"
  Bus Selector13/10 -> sSector/1  "<sSector>"
  Bus Selector34/1 -> ETotalRequested/1  "<ETotalRequested>"
  Bus Selector34/2 -> ESector1Remaining/1  "<ESector1Remaining>"
  Bus Selector34/3 -> ESector2Remaining/1  "<ESector2Remaining>"
  Bus Selector34/4 -> ESector3Remaining/1  "<ESector3Remaining>"
  Bus Selector34/5 -> ESector4Remaining/1  "<ESector4Remaining>"
  Bus Selector54/1 -> NSector9Remaining/1  "<NSector9Remaining>"
  Bus Selector54/2 -> NSector10Remaining/1  "<NSector10Remaining>"
  Bus Selector54/3 -> NSector11Remaining/1  "<NSector11Remaining>"
  Bus Selector54/4 -> NSector12Remaining/1  "<NSector12Remaining>"
  Bus Selector54/5 -> ESector5Remaining/1  "<ESector5Remaining>"
  Bus Selector54/6 -> ESector6Remaining/1  "<ESector6Remaining>"
  Bus Selector54/7 -> ESector7Remaining/1  "<ESector7Remaining>"
  Bus Selector53/1 -> ESector9Remaining/1  "<ESector9Remaining>"
  Bus Selector53/2 -> ESector10Remaining/1  "<ESector10Remaining>"
  Bus Selector53/3 -> ESector11Remaining/1  "<ESector11Remaining>"
  Bus Selector53/4 -> ESector12Remaining/1  "<ESector12Remaining>"
  Bus Selector53/5 -> NSector1Remaining/1  "<NSector1Remaining>"
  Bus Selector53/6 -> NSector2Remaining/1  "<NSector2Remaining>"
  Bus Selector38/1 -> NSectorGlobal/1  "<NSectorGlobal>"
  Bus Selector38/2 -> NSectorLap/1  "<NSectorLap>"
  Bus Selector38/3 -> NSector3Remaining/1  "<NSector3Remaining>"
  Bus Selector38/4 -> NSector4Remaining/1  "<NSector4Remaining>"
  Bus Selector38/5 -> NSector5Remaining/1  "<NSector5Remaining>"
  Bus Selector38/6 -> NSector6Remaining/1  "<NSector6Remaining>"
  Bus Selector38/7 -> NSector7Remaining/1  "<NSector7Remaining>"
  Bus Selector38/8 -> NSector8Remaining/1  "<NSector8Remaining>"
  Bus Selector38/9 -> ESector8Remaining/1  "<ESector8Remaining>"
  Bus Selector55/1 -> rTorqueSplitOW/1  "<rTorqueSplitOW>"
  Bus Selector55/2 -> PRegenMax/1  "<PRegenMax>"
  Bus Selector55/3 -> PRegenMaxEM/1  "<PRegenMaxEM>"
  Bus Selector55/4 -> PRegenMaxOW/1  "<PRegenMaxOW>"
  Bus Selector55/5 -> rTVMultiplier/1  "<rTVMultiplier>"
  Bus Selector55/6 -> rTVMultiplierEM/1  "<rTVMultiplierEM>"
  Bus Selector55/7 -> rTVMultiplierOW/1  "<rTVMultiplierOW>"
  Bus Selector55/8 -> rEngineBrakingSplit/1  "<rEngineBrakingSplit>"
  Bus Selector55/9 -> rEngineBrakingSplitEM/1  "<rEngineBrakingSplitEM>"
  Bus Selector55/10 -> rEngineBrakingSplitOW/1  "<rEngineBrakingSplitOW>"
  Bus Selector55/11 -> rSOC/1  "<rSOC>"
  Bus Selector55/12 -> BReadyToDrive/1  "<BReadyToDrive>"
  Bus Selector55/13 -> BTVOn/1  "<BTVOn>"
  Bus Selector18/9 -> NTCKdSelector/1  "<NTCKdSelector>"
  Bus Selector18/10 -> NPCKpSelector/1  "<NPCKpSelector>"
  Bus Selector18/11 -> MRegenMax/1  "<MRegenMax>"
  Bus Selector18/12 -> rTorqueSplitEM/1  "<rTorqueSplitEM>"
  Bus Selector18/8 -> EOffset/1  "<EOffset>"
  Bus Selector18/7 -> rGrip/1  "<rGrip>"
  Bus Selector18/6 -> PEngineBrakingOW/1  "<PEngineBrakingOW>"
  Bus Selector18/1 -> PDischargeMax/1  "<PDischargeMax>"
  Bus Selector18/2 -> PDischargeMaxEM/1  "<PDischargeMaxEM>"
  Bus Selector18/3 -> PDischargeMaxOW/1  "<PDischargeMaxOW>"
  Bus Selector18/4 -> PEngineBraking/1  "<PEngineBraking>"
  Bus Selector18/5 -> PEngineBrakingEM/1  "<PEngineBrakingEM>"
  [Global] -> Bus Selector11/1
  Bus Selector11/1 -> BTVOnEM/1  "<BTVOnEM>"
  Bus Selector11/2 -> BTVOnOW/1  "<BTVOnOW>"
  Bus Selector11/3 -> BDrivetrainCoolingOn/1  "<BDrivetrainCoolingOn>"
  Bus Selector11/4 -> BDrivetrainCoolingOnEM/1  "<BDrivetrainCoolingOnEM>"
  Bus Selector11/5 -> BDrivetrainCoolingOnOW/1  "<BDrivetrainCoolingOnOW>"
  Bus Selector11/6 -> BTCOn/1  "<BTCOn>"
  Bus Selector11/9 -> BEMSOn/1  "<BEMSOn>"
  Bus Selector11/10 -> BEMSOnEM/1  "<BEMSOnEM>"
  Bus Selector11/11 -> BEMSOnOW/1  "<BEMSOnOW>"
  Bus Selector11/7 -> BTCOnEM/1  "<BTCOnEM>"
  Bus Selector11/8 -> BTCOnOW/1  "<BTCOnOW>"
  Bus Selector11/12 -> BSpinningModeOn/1  "<BSpinningModeOn>"
  Bus Selector11/13 -> BSpinningModeOnEM/1  "<BSpinningModeOnEM>"
  Bus Selector11/14 -> BSpinningModeOnOW/1  "<BSpinningModeOnOW>"
  Bus Selector11/15 -> rSOE/1  "<rSOE>"
  Bus Selector11/16 -> BBalancingOnOut/1  "<BBalancingOn>"
  Bus Selector11/17 -> BBMSP0A0COut/1  "<BBMSP0A0C>"
  Bus Selector11/18 -> BBMSP0A0EOut/1  "<BBMSP0A0E>"
  Bus Selector11/19 -> BBMSP0A10Out/1  "<BBMSP0A10>"
  Bus Selector11/20 -> BBMSP0A80Out/1  "<BBMSP0A80>"
  Bus Selector11/21 -> BBMSP0AC0Out/1  "<BBMSP0AC0>"
  Bus Selector11/23 -> NLap/1  "<NLap>"
  Bus Selector11/22 -> BBMSP0AFAOut/1  "<BBMSP0AFA>"
  Bus Selector11/24 -> NEventMode/1  "<NEventMode>"
  Bus Selector24/4 -> MTractionControlRLTotal/1  "<MTractionControlRLTotal>"
  Bus Selector24/6 -> MTractionControlFLTotal/1  "<MTractionControlFLTotal>"
  Bus Selector11/25 -> rTorqueSplit/1  "<rTorqueSplit>"
  Bus Selector11/26 -> NThrottleMap/1  "<NThrottleMap>"
  Bus Selector11/28 -> NThrottleMapOW/1  "<NThrottleMapOW>"
  Bus Selector11/27 -> NThrottleMapEM/1  "<NThrottleMapEM>"
  Bus Selector7/1 -> NInvDTCRLOut/1  "<NInvDTCRL>"
  Bus Selector7/2 -> NInvDTCRROut/1  "<NInvDTCRR>"
  Bus Selector7/3 -> NInvDTCFLOut/1  "<NInvDTCFL>"
  Bus Selector7/4 -> NInvDTCFROut/1  "<NInvDTCFR>"
  Bus Selector2/7 -> BQuitInvOnRLCAN3/1  "<BQuitInvOnRL>"
  Bus Selector2/8 -> BQuitInvOnFLCAN3/1  "<BQuitInvOnFL>"
  Bus Selector2/9 -> BQuitInvOnRRCAN3/1  "<BQuitInvOnRR>"
  Bus Selector2/10 -> BQuitInvOnFRCAN3/1  "<BQuitInvOnFR>"
  Bus Selector2/11 -> BInvErrorResetRLCAN3/1  "<BInvErrorResetRL>"
  Bus Selector2/12 -> BInvErrorResetRRCAN3/1  "<BInvErrorResetRR>"
  Bus Selector2/13 -> BInvErrorResetFLCAN3/1  "<BInvErrorResetFL>"
  Bus Selector2/14 -> BInvErrorResetFRCAN3/1  "<BInvErrorResetFR>"
  Digital Port Read1/1 -> NOT4/1
  NOT4/1 -> Digital Port Write/1, CAN Rx/Enable
  Etas_Signals_13/1 -> Bus Selector27/1
  Bus Selector26/4 -> CAN Tx11/5(rInvTemperatureDerateRL)  "<rInvTemperatureDerateRL>"
  Bus Selector17/13 -> CAN Tx1/14(rSOCRegenDerate)  "<rSOCRegenDerate>"
  Bus Selector56/1 -> CAN Tx9/2(MSpinningModelRL)  "<MSpinningModelRL>"
  Bus Selector50/2 -> CAN Tx6/3(BBalancingActive)  "<BBalancingActive>"
  Bus Selector41/5 -> CAN Tx2/6(vWheelRL)  "<vWheelRL>"
  Bus Selector45/6 -> CAN Tx5/7(NTractionControlMultiplierRR)  "<NTractionControlMultiplierRR>"
  Bus Selector28/4 -> CAN Tx13/5(MDriverDischargeRequested)  "<MDriverDischargeRequested>"
  Bus Selector50/6 -> CAN Tx6/7(MTractionControlRRTotal)  "<MTractionControlRRTotal>"
  Bus Selector44/9 -> CAN Tx3/10(PPowerControllerRequested)  "<PPowerControllerRequested>"
  Bus Selector17/12 -> CAN Tx1/13(rSOCDischargeDerate)  "<rSOCDischargeDerate>"
  Bus Selector43/2 -> CAN Tx19/3(BBrakeLightOnRequest)  "<BBrakeLight>"
  Bus Selector39/4 -> CAN Tx17/6(VCellMin)  "<VCellMin>"
  Bus Selector44/2 -> CAN Tx3/3(BBrakeError)  "<BBrakeError>"
  Bus Selector28/6 -> CAN Tx13/7(MFRFinal)  "<MFRFinal>"
  Bus Selector41/6 -> CAN Tx2/7(vWheelRR)  "<vWheelRR>"
  Bus Selector26/6 -> CAN Tx11/7(rMotorTemperatureDerateFL)  "<rMotorTemperatureDerateFL>"
  Bus Selector26/8 -> CAN Tx11/9(rMotorTemperatureDerateRL)  "<rMotorTemperatureDerateRL>"
  Etas_Signals_06/1 -> Bus Selector45/1
  Bus Selector51/4 -> CAN Tx7/5(MTorqueVectoringFR)  "<MTorqueVectoringFR>"
  Etas_Signals_17/1 -> Bus Selector37/1
  Bus Selector40/4 -> CAN Tx18/5(rRegenPaddle)  "<rRegenPaddle>"
  From52/1 -> CAN Tx2/1(MCPInitialized)
  Bus Selector50/4 -> CAN Tx6/5(MTractionControlFRTotal)  "<MTractionControlFRTotal>"
  From63/1 -> CAN Tx12/1(MCPInitialized)
  Bus Selector26/1 -> CAN Tx11/2(MTotalEMSRequested)  "<MTotalEMSRequested>"
  Bus Selector50/3 -> CAN Tx6/4(MTractionControlFLTotal)  "<MTractionControlFLTotal>"
  Bus Selector44/3 -> CAN Tx3/4(BBrakeOn)  "<BBrakeOn>"
  SPI Controller Transfer3/1 -> Terminator4/1
  Bus Selector43/5 -> CAN Tx19/6(Other)  "<BAccumulatorFanDuty>"
  Bus Selector41/3 -> CAN Tx2/4(vWheelFL)  "<vWheelFL>"
  Bus Selector44/1 -> CAN Tx3/2(BAppsOk)  "<BAppsOK>"
  Bus Selector52/7 -> CAN Tx8/8(rSlipRatioOptimal)  "<rSlipRatioOptimal>"
  Bus Selector37/5 -> CAN Tx16/6(IIVTS)  "<IIVTS>"
  Bus Selector46/10 -> CAN Tx4/12(rSOC)  "<rSOC>"
  Bus Selector46/11 -> CAN Tx4/13(rSOE)  "<rSOE>"
  Bus Selector46/9 -> CAN Tx4/11(PRegen)  "<PRegen>"
  Bus Selector50/1 -> CAN Tx6/2(BBMSP0A0C)  "<BBMSP0A0C>"
  Bus Selector39/5 -> CAN Tx17/7(VLVSystem)  "<VLVSystem>"
  Bus Selector27/4 -> CAN Tx12/5(nMotorRR)  "<nMotorRR>"
  From55/1 -> CAN Tx5/1(MCPInitialized)
  Counter Free-Running/1 -> Data Type Conversion/1
  Bus Selector32/10 -> CAN Tx14/12(TMotorRR)  "<TMotorRR>"
  From65/1 -> CAN Tx14/1(MCPInitialized)
  Bus Selector28/5 -> CAN Tx13/6(MFLFinal)  "<MFLFinal>"
  Bus Selector32/6 -> CAN Tx14/8(TMotorFL)  "<TMotorFL>"
  Bus Selector45/4 -> CAN Tx5/5(NThrottleMap)  "<NThrottleMap>"
  Bus Selector16/5 -> CAN Tx/6(MTotalFinal)  "<MTotalFinal>"
  SPI Controller Transfer5/1 -> Terminator6/1
  Bus Selector51/2 -> CAN Tx7/3(BBMSP0A10)  "<BBMSP0A10>"
  Etas_Signals_19/1 -> Bus Selector40/1
  Bus Selector36/2 -> CAN Tx15/3(NInvDTCFR)  "<NInvDTCFR>"
  Bus Selector16/9 -> CAN Tx/10(VChassis)  "<vChassis>"
  Bus Selector56/4 -> CAN Tx9/5(MTorqueDistributionFR)  "<MTorqueDistributionFR>"
  Bus Selector32/7 -> CAN Tx14/9(TMotorFR)  "<TMotorFR>"
  Bus Selector17/6 -> CAN Tx1/7(rHighCellTempDischargeDerate)  "<rHighCellTemperatureDischargeDerate>"
  Bus Selector46/8 -> CAN Tx4/10(PEngineBraking)  "<PEngineBraking>"
  Bus Selector52/5 -> CAN Tx8/6(MSpinningModelFR)  "<MSpinningModelFR>"
  Bus Selector45/3 -> CAN Tx5/4(NABSMultiplierRR)  "<NABSMultiplierRR>"
  Multiplexer?/1 -> CAN Tx4/2(Multiplexer05)
  Bus Selector17/14 -> CAN Tx1/15(rSOCTargetError)  "<rSOCTargetError>"
  Bus Selector16/6 -> CAN Tx/7(PActual)  "<PActual>"
  Bus Selector32/1 -> CAN Tx14/3(TInvFL)  "<TInvFL>"
  Bus Selector44/11 -> CAN Tx3/12(tBrakeError)  "<tBrakeError>"
  From61/1 -> CAN Tx10/1(MCPInitialized)
  Subsystem/1(MCPInitialized) -> [MCPInitialized]
  Bus Selector36/1 -> CAN Tx15/2(NInvDTCFL)  "<NInvDTCFL>"
  Bus Selector52/1 -> CAN Tx8/2(MDischargeLimited)  "<MDischargeLimited>"
  From62/1 -> CAN Tx11/1(MCPInitialized)
  Bus Selector37/7 -> CAN Tx16/8(VCDAccu)  "<VDCAccumulator>"
  Bus Selector17/2 -> CAN Tx1/3(BBMSP0AC0)  "<BBMSP0AC0>"
  Bus Selector51/3 -> CAN Tx7/4(MTorqueVectoringFL)  "<MTorqueVectoringFL>"
  Bus Selector17/9 -> CAN Tx1/10(rLowCellVoltageDischargeDerate)  "<rLowCellVoltageDischargeDerate>"
  Bus Selector51/1 -> CAN Tx7/2(BBMSP0A0E)  "<BBMSP0A0E>"
  Bus Selector25/2 -> CAN Tx10/4(VDamperPotentiometerRR)  "<VDamperPotentiometerFR>"
  Etas_Signals_05/1 -> Bus Selector46/1
  Bus Selector50/5 -> CAN Tx6/6(MTractionControlRLTotal)  "<MTractionControlRLTotal>"
  Bus Selector43/1 -> CAN Tx19/2(BAccumulatorFanOnRequest)  "<BAccumulatorFanOn>"
  Bus Selector50/7 -> CAN Tx6/8(NABSMultiplierFL)  "<NABSMultiplierFL>"
  Constant1/1 -> CAN Tx17/8(tEtasOn)
  Bus Selector37/8 -> CAN Tx16/9(VCDInvRL)  "<VDCInvRL>"
  PDM_Req/1 -> Bus Selector43/1
  From56/1 -> CAN Tx6/1(MCPInitialized)
  Bus Selector45/5 -> CAN Tx5/6(NTractionControlMultiplierRL)  "<NTractionControlMultiplierRL>"
  From51/1 -> CAN Tx1/1(MCPInitialized)
  RTS1/1 -> SPI Controller Transfer2/1
  Bus Selector17/5 -> CAN Tx1/6(rDischargeDerate)  "<rDischargeDerate>"
  Bus Selector25/1 -> CAN Tx10/3(VDamperPotentiometerRL)  "<VDamperPotentiometerFL>"
  Etas_Signals_16/1 -> Bus Selector36/1
  Bus Selector46/7 -> CAN Tx4/9(NTorqueSplitSpeedSelector)  "<NTorqueSplitSpeedSelector>"
  Bus Selector16/2 -> CAN Tx/3(BEncoderErrorRear)  "<BEncoderErrorRear>"
  From54/1 -> CAN Tx4/1(MCPInitialized)
  Bus Selector56/5 -> CAN Tx9/6(MTorqueDistributionRL)  "<MTorqueDistributionRL>"
  Bus Selector16/7 -> CAN Tx/8(PPowerControllerProportionalTerm)  "<PPowerControllerProportionalTerm>"
  Bus Selector44/8 -> CAN Tx3/9(MPowerControllerRequested)  "<MPowerControllerRequested>"
  Bus Selector56/2 -> CAN Tx9/3(MSpinningModelRR)  "<MSpinningModelRR>"
  Data Type Conversion/1 -> CAN Tx10/2(TEST_NUMBER)
  SPI Controller Transfer2/1 -> Terminator3/1
  Bus Selector40/1 -> CAN Tx18/2(PDischargeLimited)  "<PDischargeLimited>"
  Bus Selector45/1 -> CAN Tx5/2(BReadyToDrive)  "<BReadyToDrive>"
  Etas_Signals_14/1 -> Bus Selector28/1
  Bus Selector17/8 -> CAN Tx1/9(rInvTemperatureDerate)  "<rInvTemperatureDerate>"
  Bus Selector39/2 -> CAN Tx17/3(TCellMin)  "<TCellMin>"
  Bus Selector56/6 -> CAN Tx9/7(MTorqueDistributionRR)  "<MTorqueDistributionRR>"
  From60/1 -> CAN Tx9/1(MCPInitialized)
  From70/1 -> CAN Tx19/1(MCPInitialized)
  Bus Selector32/5 -> CAN Tx14/7(TInvRR)  "<TInvRR>"
  Bus Selector52/2 -> CAN Tx8/3(MDriverRegenRequested)  "<MDriverRegenRequested>"
  Bus Selector16/3 -> CAN Tx/4(BSpinningModelActivated)  "<BSpinningModelActivated>"
  Bus Selector32/8 -> CAN Tx14/10(TMotorMax)  "<TMotorMax>"
  Bus Selector45/7 -> CAN Tx5/8(rSlipRatioFLActual)  "<rSlipRatioFLActual>"
  Etas_Signals_04/1 -> Bus Selector44/1
  Bus Selector40/5 -> CAN Tx18/6(rSplitRear)  "<rSplitRear>"
  Bus Selector52/3 -> CAN Tx8/4(MRegenLimited)  "<MRegenLimited>"
  Bus Selector45/2 -> CAN Tx5/3(NABSMultiplierRL)  "<NABSMultiplierRL>"
  Bus Selector46/4 -> CAN Tx4/6(NModeNumberDisplay5)  "<NModeNumberDisplay5>"
  Bus Selector32/4 -> CAN Tx14/6(TInvRL)  "<TInvRL>"
  Bus Selector17/15 -> CAN Tx1/16(rSpeedRegenDerate)  "<rSpeedRegenDerate>"
  From57/1 -> CAN Tx/1(MCPInitialized)
  Bus Selector26/3 -> CAN Tx11/4(rInvTemperatureDerateFR)  "<rInvTemperatureDerateFR>"
  Bus Selector26/5 -> CAN Tx11/6(rInvTemperatureDerateRR)  "<rInvTemperatureDerateRR>"
  Bus Selector27/2 -> CAN Tx12/3(nMotorFR)  "<nMotorFR>"
  From69/1 -> CAN Tx18/1(MCPInitialized)
  Bus Selector32/3 -> CAN Tx14/5(TInvMax)  "<TInvMax>"
  Bus Selector43/4 -> CAN Tx19/5(BReadyToDriveBuzzerRequest)  "<BReadyToDriveBuzzer>"
  Bus Selector17/1 -> CAN Tx1/2(BBMSP0A80)  "<BBMSP0A80>"
  Bus Selector46/6 -> CAN Tx4/8(NPowerControllerKpSelector)  "<NPowerControllerKpSelector>"
  From68/1 -> CAN Tx17/1(MCPInitialized)
  Bus Selector17/4 -> CAN Tx1/5(PDischarge)  "<PDischarge>"
  Bus Selector44/5 -> CAN Tx3/6(BRegenOn)  "<BRegenOn>"
  Bus Selector37/2 -> CAN Tx16/3(BEMSActivated)  "<BEMSActivated>"
  Bus Selector16/4 -> CAN Tx/5(BTorqueVectoringOk)  "<BTorqueVectoringOK>"
  Etas_Signals_03/1 -> Bus Selector41/1
  Bus Selector45/9 -> CAN Tx5/10(rSlipRatioRLActual)  "<rSlipRatioRLActual>"
  From64/1 -> CAN Tx13/1(MCPInitialized)
  Bus Selector56/3 -> CAN Tx9/4(MTorqueDistributionFL)  "<MTorqueDistributionFL>"
  Bus Selector51/7 -> CAN Tx7/8(NTractionControlMultiplierFL)  "<NTractionControlMultiplierFL>"
  Bus Selector28/2 -> CAN Tx13/3(BEMS1000mPoint)  "<BEMS1000mPoint>"
  From58/1 -> CAN Tx7/1(MCPInitialized)
  Bus Selector41/1 -> CAN Tx2/2(rSOETargetError)  "<rSOETargetError>"
  Bus Selector17/3 -> CAN Tx1/4(BBMSP0AFA)  "<BBMSP0AFA>"
  Bus Selector44/6 -> CAN Tx3/7(BThrottleError)  "<BThrottleError>"
  Bus Selector17/7 -> CAN Tx1/8(rHighCellTempRegenDerate)  "<rHighCellTemperatureRegenDerate>"
  Bus Selector51/6 -> CAN Tx7/7(MTorqueVectoringRR)  "<MTorqueVectoringRR>"
  Bus Selector32/9 -> CAN Tx14/11(TMotorRL)  "<TMotorRL>"
  Bus Selector45/8 -> CAN Tx5/9(rSlipRatioFRActual)  "<rSlipRatioFRActual>"
  From67/1 -> CAN Tx16/1(MCPInitialized)
  Bus Selector37/1 -> CAN Tx16/2(BAccumulatorFanOn)  "<BAccumulatorFanOn>"
  Bus Selector17/10 -> CAN Tx1/11(rMotorTemperatureDerate)  "<rMotorTemperatureDerate>"
  Bus Selector40/2 -> CAN Tx18/3(aSteeringAngle)  "<aSteeringAngle>"
  RTS4/1 -> SPI Controller Transfer5/1
  Bus Selector37/4 -> CAN Tx16/5(IBMSHallEffect)  "<IBMSHallEffect>"
  Bus Selector43/3 -> CAN Tx19/4(BInvLVOnRequest)  "<BInvLVOn>"
  Bus Selector17/11 -> CAN Tx1/12(rRegenDerate)  "<rRegenDerate>"
  Bus Selector40/7 -> CAN Tx18/8(tPedalOverlap)  "<tPedalOverlap>"
  Bus Selector16/1 -> CAN Tx/2(BEncoderErrorFront)  "<BEncoderErrorFront>"
  Bus Selector28/8 -> CAN Tx13/9(MRRFinal)  "<MRRFinal>"
  Etas_Signals_10/1 -> Bus Selector56/1
  Bus Selector26/10 -> CAN Tx11/11(rThrottlePedal1)  "<rThrottlePedal>"
  RTS2/1 -> SPI Controller Transfer3/1
  Etas_Signals_02/1 -> Bus Selector17/1
  Bus Selector46/13 -> CAN Tx4/15(sChassis)  "<sChassis>"
  Bus Selector46/12 -> CAN Tx4/14(rTorqueVectoringMultiplier)  "<rTorqueVectoringMultiplier>"
  Multiplexer1?/1 -> CAN Tx14/2(Multiplexer15)
  Bus Selector44/4 -> CAN Tx3/5(BPedalOverlap)  "<BPedalOverlap>"
  Bus Selector36/3 -> CAN Tx15/4(NInvDTCRL)  "<NInvDTCRL>"
  Bus Selector26/7 -> CAN Tx11/8(rMotorTemperatureDerateFR)  "<rMotorTemperatureDerateFR>"
  Bus Selector51/5 -> CAN Tx7/6(MTorqueVectoringRL)  "<MTorqueVectoringRL>"
  Bus Selector40/3 -> CAN Tx18/4(nYawRateErrorActual)  "<nYawRateErrorActual>"
  Bus Selector37/6 -> CAN Tx16/7(MTotalRequested)  "<MTotalRequested>"
  From59/1 -> CAN Tx8/1(MCPInitialized)
  Bus Selector26/9 -> CAN Tx11/10(rMotorTemperatureDerateRR)  "<rMotorTemperatureDerateRR>"
  Etas_Signals_08/1 -> Bus Selector51/1
  Bus Selector36/6 -> CAN Tx15/7(VCellDelta)  "<VCellDelta>"
  Bus Selector50/8 -> CAN Tx6/9(NABSMultiplierFR)  "<NABSMultiplierFR>"
  From53/1 -> CAN Tx3/1(MCPInitialized)
  Bus Selector52/6 -> CAN Tx8/7(NCarState)  "<NCarState>"
  Etas_Signals_09/1 -> Bus Selector52/1
  Bus Selector27/1 -> CAN Tx12/2(nMotorFL)  "<nMotorFL>"
  Constant/1 -> CAN Tx17/4(TEtas)
  Bus Selector28/3 -> CAN Tx13/4(BEMS995mPoint)  "<BEMS995mPoint>"
  Bus Selector39/3 -> CAN Tx17/5(VCellMax)  "<VCellMax>"
  Etas_Signals_07/1 -> Bus Selector50/1
  Bus Selector41/2 -> CAN Tx2/3(sEMS1000m)  "<sEMS1000m>"
  Etas_Signals_15/1 -> Bus Selector32/1
  Bus Selector26/2 -> CAN Tx11/3(rInvTemperatureDerateFL)  "<rInvTemperatureDerateFL>"
  Bus Selector41/4 -> CAN Tx2/5(vWheelFR)  "<vWheelFR>"
  Bus Selector52/4 -> CAN Tx8/5(MSpinningModelFL)  "<MSpinningModelFL>"
  Bus Selector46/2 -> CAN Tx4/4(NBMSState)  "<NBMSState>"
  Bus Selector44/12 -> CAN Tx3/13(tThrottleError)  "<tThrottleError>"
  Etas_Signals_11/1 -> Bus Selector25/1
  Bus Selector36/4 -> CAN Tx15/5(NInvDTCRR)  "<NInvDTCRR>"
  Bus Selector44/10 -> CAN Tx3/11(rThrottlePedal)  "<rThrottlePedal>"
  Etas_Signals_18/1 -> Bus Selector39/1
  Bus Selector39/1 -> CAN Tx17/2(NTractionControlKpSelector)  "<NTractionControlKpSelector>"
  Bus Selector28/7 -> CAN Tx13/8(MRLFinal)  "<MRLFinal>"
  Bus Selector45/10 -> CAN Tx5/11(rSlipRatioRRActual)  "<rSlipRatioRRActual>"
  Bus Selector46/5 -> CAN Tx4/7(NModeNumberDisplay6)  "<NModeNumberDisplay6>"
  Bus Selector36/5 -> CAN Tx15/6(TCellMax)  "<TCellMax>"
  Etas_Signals_01/1 -> Bus Selector16/1
  Bus Selector40/6 -> CAN Tx18/7(tAppsTimer)  "<tAppsTimer>"
  Bus Selector46/3 -> CAN Tx4/5(NInvState)  "<NInvState>"
  Bus Selector32/2 -> CAN Tx14/4(TInvFR)  "<TInvFR>"
  Bus Selector51/8 -> CAN Tx7/9(NTractionControlMultiplierFR)  "<NTractionControlMultiplierFR>"
  Bus Selector16/8 -> CAN Tx/9(PPowerControllerIntegralTerm)  "<PPowerControllerIntegralTerm>"
  From66/1 -> CAN Tx15/1(MCPInitialized)
  Etas_Signals_12/1 -> Bus Selector26/1
  Bus Selector44/7 -> CAN Tx3/8(BTorqueVectoringActivated)  "<BTorqueVectoringActivated>"
  Bus Selector37/3 -> CAN Tx16/4(BTractionControlActivated)  "<BTractionControlActivated>"
  Bus Selector27/3 -> CAN Tx12/4(nMotorRL)  "<nMotorRL>"
  Bus Selector28/1 -> CAN Tx13/2(BDischargeAllowed)  "<BDischargeAllowed>"
  Bus Selector46/1 -> CAN Tx4/3(NBMSDLC)  "<NBMSDLC>"
  Compare To Constant/1 -> ?
  Counter Limited/1 -> Compare To Constant/1
  Bus Creator2/1 -> [DDU7]
  CAN Rx/5(VBrakeR) -> Bus Creator2/6  "VBrakeR"
  CAN Rx/1(VSteeringAngle) -> Bus Creator2/2  "VSteeringAngle"
  CAN Rx/4(VBrakeF) -> Bus Creator2/5  "VBrakeF"
  CAN Rx/3(VThrottlePedal2) -> Bus Creator2/4  "VThrottlePedal2"
  CAN Rx/6(VDamperPotentiometerFR) -> Bus Creator2/7  "VDamperPotentiometerFR"
  CAN Rx/2(VThrottlePedal1) -> Bus Creator2/3  "VThrottlePedal1"
  CAN Rx/7(VDamperPotentiometerFL) -> Bus Creator2/8  "VDamperPotentiometerFL"
  CAN Rx/8(vLateralIMU) -> Bus Creator3/1  "vLateralIMU"
  CAN Rx/11(gLateralIMU) -> Bus Creator3/4  "gLateralIMU"
  CAN Rx/10(vLongitudinalIMU) -> Bus Creator3/3  "vLongitudinalIMU"
  Bus Creator3/1 -> [IMU]
  CAN Rx/9(gVerticalIMU) -> Bus Creator3/2  "gVerticalIMU"
  CAN Rx/13(nYawRateIMU) -> Bus Creator3/6  "nYawRateIMU"
  CAN Rx/12(gLongitudingalIMU) -> Bus Creator3/5
  CAN Rx/21(NPageSelectRotary) -> Bus Creator4/5  "NPageSelectRotary"
  CAN Rx/17(BSteeringWheelButton1) -> Digital Port Write1/1, CAN Tx20/2(BDischargeAllowed), Bus Creator4/1  "BSteeringWheelButton1"
  CAN Rx/19(BSteeringWheelButton3) -> Bus Creator4/3, CAN Tx20/4(BThrottleError)  "BSteeringWheelButton3"
  CAN Rx/24(VRegenPaddle1) -> Bus Creator4/8  "VRegenPaddle1"
  CAN Rx/23(NEventModeRotary) -> Bus Creator4/7  "NEventModeRotary"
  CAN Rx/22(NParameterRotary) -> Bus Creator4/6  "NParameterRotary"
  CAN Rx/18(BSteeringWheelButton2) -> Bus Creator4/2, CAN Tx20/3(BBrakeError)  "BSteeringWheelButton2"
  CAN Rx/20(BSteeringWheelButton4) -> Bus Creator4/4  "BSteeringWheelButton4"
  CAN Rx/25(VRegenPaddle2) -> Bus Creator4/9  "VRegenPaddle2"
  Bus Creator4/1 -> [STW]
  CAN Rx/16(nRollIMU) -> Terminator/1
  CAN Rx/14(gSlipIMU) -> Terminator2/1
  CAN Rx/15(nPitchIMU) -> Terminator1/1
  Constant2/1 -> Bus Creator2/1
  [MCPInitialized] -> CAN Tx20/1(MCPInitialized)
  Unit Delay/1 -> NOT/1
  NOT/1 -> Unit Delay/1
  Constant3/1 -> CAN Tx20/10(PActual), CAN Tx20/11(MRRFinal), CAN Tx20/9(MFRFinal), CAN Tx20/8(MRLFinal), CAN Tx20/7(IVTSOut), CAN Tx20/6(MFLFinal), CAN Tx20/5(BOverpower)
  SPI Controller Transfer1/1 -> Terminator5/1
  RTS3/1 -> SPI Controller Transfer1/1
  CAN Rx/26(ID) -> CAN Tx20/12(Number1)
  CAN Rx/27(Length) -> CAN Tx20/13(Number2)
